simulink model "plant_n"  (R2023a)
settings: Solver=FixedStepAuto  StartTime=0.0  StopTime=200  FixedStep=0.01  RelTol=1e-3
values from neighbouring files (symbols this model uses):
  filter_3 = conv([0.1,1],conv([0.1 1],[0.1 1]))    [main_proj.m]
  filter_x = conv([0.7,1],conv([0.7 1],[0.7 1]))    [main_proj.m]
  kd = 1.117    [main_proj.m]
  ki = 4.47    [main_proj.m]
  kp = 5.366    [main_proj.m]
libraries: neural x772, slpidlib x6
(part 1 of 26)
settings Model: Creator=Alex  LastModifiedBy=Alex

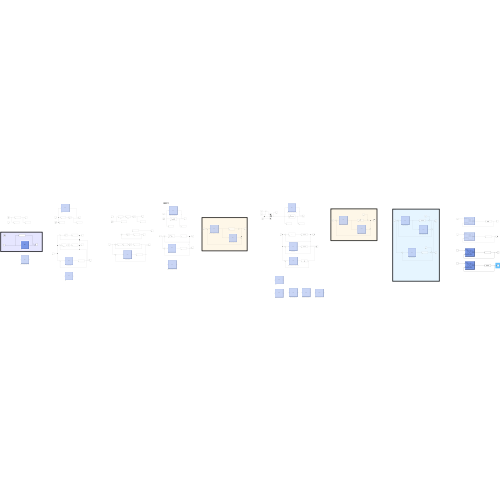
[thumbnail: Simulink's stored preview of the top-level diagram]
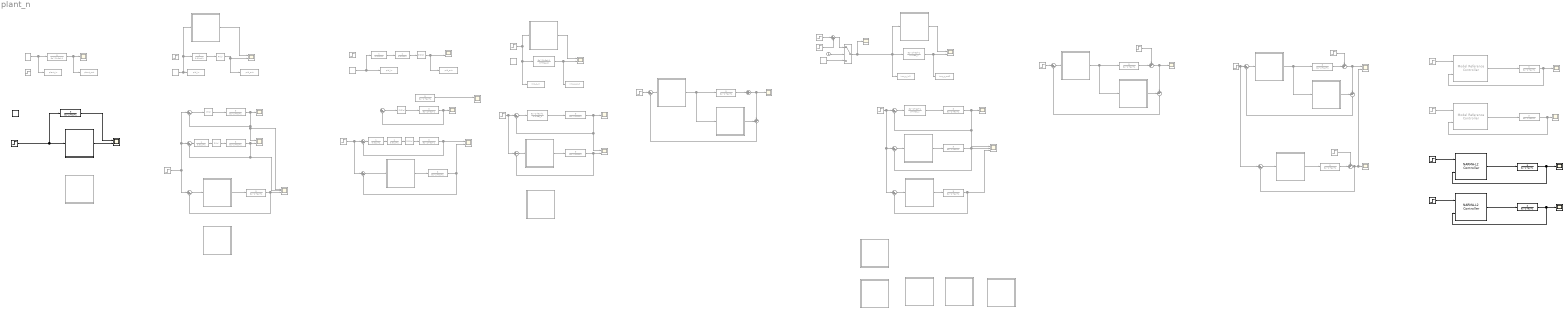
== system plant_n ==
  note: IMC1
  note: IMC1
  note: #2-3
  note: IMC2
  note: Compare
  Clock : Clock  Commented=on
  Filter{,1..5} (6 alike) : TransferFcn  Commented=on  Denominator=[0.01 1]
  Hr2 Neural Network : Subsystem  Commented=on  mask{pi_input_1_delayed_1=0, pi_input_1_delayed_2=0, pi_input_1_delayed_3=0, pi_input_1_delayed_4=0, pi_input_1_delayed_5=0, pi_input_1_delayed_6=0, ai_layer_2_delayed_1=0, ai_layer_2_delayed_2=0, ai_layer_2_delayed_3=0, ai_layer_2_delayed_4=0, ai_layer_2_delayed_5=0, ai_layer_2_delayed_6=0}
      mask prompts: pi_input_1_delayed_1 "Preprocessed initial input 1 state at timestep 0."; pi_input_1_delayed_2 "Preprocessed initial input 1 state at timestep -1."; pi_input_1_delayed_3 "Preprocessed initial input 1 state at timestep -2."; pi_input_1_delayed_4 "Preprocessed initial input 1 state at timestep -3."; pi_input_1_delayed_5 "Preprocessed initial input 1 state at timestep -4."; pi_input_1_delayed_6 "Preprocessed initial input 1 state at timestep -5."; ai_layer_2_delayed_1 "Initial layer 2 state at timestep 0."; ai_layer_2_delayed_2 "Initial layer 2 state at timestep -1."; ai_layer_2_delayed_3 "Initial layer 2 state at timestep -2."; ai_layer_2_delayed_4 "Initial layer 2 state at timestep -3."; ai_layer_2_delayed_5 "Initial layer 2 state at timestep -4."; ai_layer_2_delayed_6 "Initial layer 2 state at timestep -5."
      mask help: NARX Neural Network
      mask Display: e = 0.06;c1 = [120 150 230]/255;c2 = ([120 150 230]+0)/383;c3 = ([120 150 230]+128)/383;patch([0 1 1 0],[0 0 1 1],c1);patch([0 1 1 1-e 1-e 0+e],[0 0 1 1-e 0+e 0+e],c2);patch([0 0 1 1-e 0+e 0+e],[0 1 1 1-e 1-e 0+e],c3);plot([0 1 1 0 0],[0 0 1 1 0]);fprintf('NNET');port_label('input',1,' x');port_label('output',1,'y ');
  Hr2 Neural Network1 : Subsystem  Commented=on  mask{pi_input_1_delayed_1=0, pi_input_1_delayed_2=0, pi_input_1_delayed_3=0, pi_input_1_delayed_4=0, pi_input_1_delayed_5=0, pi_input_1_delayed_6=0, ai_layer_2_delayed_1=0, ai_layer_2_delayed_2=0, ai_layer_2_delayed_3=0, ai_layer_2_delayed_4=0, ai_layer_2_delayed_5=0, ai_layer_2_delayed_6=0}
      mask prompts: pi_input_1_delayed_1 "Preprocessed initial input 1 state at timestep 0."; pi_input_1_delayed_2 "Preprocessed initial input 1 state at timestep -1."; pi_input_1_delayed_3 "Preprocessed initial input 1 state at timestep -2."; pi_input_1_delayed_4 "Preprocessed initial input 1 state at timestep -3."; pi_input_1_delayed_5 "Preprocessed initial input 1 state at timestep -4."; pi_input_1_delayed_6 "Preprocessed initial input 1 state at timestep -5."; ai_layer_2_delayed_1 "Initial layer 2 state at timestep 0."; ai_layer_2_delayed_2 "Initial layer 2 state at timestep -1."; ai_layer_2_delayed_3 "Initial layer 2 state at timestep -2."; ai_layer_2_delayed_4 "Initial layer 2 state at timestep -3."; ai_layer_2_delayed_5 "Initial layer 2 state at timestep -4."; ai_layer_2_delayed_6 "Initial layer 2 state at timestep -5."
      mask help: NARX Neural Network
      mask Display: e = 0.06;c1 = [120 150 230]/255;c2 = ([120 150 230]+0)/383;c3 = ([120 150 230]+128)/383;patch([0 1 1 0],[0 0 1 1],c1);patch([0 1 1 1-e 1-e 0+e],[0 0 1 1-e 0+e 0+e],c2);patch([0 0 1 1-e 0+e 0+e],[0 1 1 1-e 1-e 0+e],c3);plot([0 1 1 0 0],[0 0 1 1 0]);fprintf('NNET');port_label('input',1,' x');port_label('output',1,'y ');
  Model Reference Controller : neural/Control Systems/Model Reference Controller  Commented=on  Nrc=2  Nic=1  Njc=2  IW_y=[1.3296070716326384709 -0.36667365564127274435;-0.92185323515790129623 0.32176549306151730478;1.8261953391711005512 1.1281754253248745812;2.081392820408017208 2.4865299205213595712;-1.4909287274670399714 0.11639212606746167367;0.46823572131003837749 0.088058028945422958667;-3.7167881282734223092 -3.6115499799353769639;1.4818494564283275494 2.7065106913308607517;1.6336147121001232119 0.5526617491453283959;-1.4099156717193841448 1.1569049865994305293;2.3686870848592893601 0.25288849028859083923;2.2287742825271403824 1.4983710960221059416;-0.99597562651575011206 0.092697495980983160568]  IW_u=[1.4743410646594798941;-0.73002540571032126238;-3.0820427704285724424;0.53364081831524945443;1.3844574682777242014;2.2994849637659218189;2.6080515112590818561;3.3191492457743909661;1.1600250344356883847;-0.81107387337725145304;-1.7263490679486648283;1.3637884727556424114;3.5961364066710643783]  IW_r=[0.45584496253579021019 0.013979066064819245518;-0.83540458064475398015 1.3369817271325503683;-0.49045911110561435375 -0.06578369498370542634;0.44086030026716438446 1.2365458882040423205;0.69033400334907890628 2.4098721877448441298;1.5039634381991009437 0.51175229301770042145;1.9013613732802914225 1.6718666996047224504;-2.9483143371280129408 -1.2964596974028812504;-0.71195000730611490702 0.54602009870251633217;0.44073655635966751953 0.35072389102907663982;-1.2261650136974546754 1.134551000123763087;2.5679363865125237609 -0.10987449572256477448;2.2584822906744599358 -0.46293788513520239825]  B1_c=[-2.6017037059917864639;2.4831616770785935877;-0.69967804536117750303;1.8461053910394569222;2.0936927854540310356;-0.65037824755168882618;-2.2310647260244911294;-0.56723571538320094465;1.5155600736459127198;-1.1274619690803939775;1.1420008123431555358;1.7485537141513041171;-0.14304865642348835175]  B2_c=0.49859367527745002135  LW_c=[-0.21560786427349326599 0.42218755085198778065 -2.5168500644863760485 -4.3042775398034240908 3.0736528575785957429 1.2004145740052258873 4.8803098890969769386 -4.903765247557268836 -2.0021893479913686065 1.1830173515845407994 1.0326255901814056504 -3.0305678461035592264 3.5511257763553163436]  retraining_c=30  max_i_int=0.3  min_i_int=0.01  max_r_int=0.3  min_r_int=0.01  Ts=0.01  S1=15  Ni=7  Nj=7  sim_file=plant_daq  trainfun=trainlm  Use_validation=1  Use_Testing=1  Use_Inc_training=0  Use_previous_weights=1  max_i=11  min_i=-11  max_r=1  min_r=-1  sam_training=7000  sam_training_c=7000  epochs=1000  epochs_c=1000  minp=-10.988507742147215041  maxp=10.979768684749934948  mint=-3.8286854023162479876  maxt=10.979768684749934948  Normalize=0  IW=[-0.096196767151805792628 0.069688900253981111987 -0.11414632395728388503 0.03380310834462384173 -0.10394306603562472602 0.050369638603738324523 -0.20070416107256491833;0.085825298980490752343 -0.13125992720494794597 0.36917943697583388563 -0.19267163875602047463 -0.12007252442864312092 -0.24919086144928226378 0.30995091781594286129;-0.12454285491314218137 -0.18617550753854025802 0.18540473952509214928 0.20790267007548821065 -0.35324104140001583163 -0.16301940699644387744 0.091419463919828858334;-5.5119777850224693555e-06 -4.3359379370616243346e-06 -1.692030312561132975e-05 -2.2407042060184435114e-06 -3.0824615230320695153e-06 -5.1366564063586963562e-06 1.6545291798370634416e-05;0.0096957497798623153845 0.38050449051489737551 0.49944098399193459503 0.052421264870644052047 0.027626071015783241341 -0.36332086427729193279 0.46254873826058989783;-3.8688801806231596213e-06 -1.0783090112052266869e-05 -1.5675682343423281539e-05 -7.4352360639534707218e-06 -5.9748050151522376945e-07 6.9622726526791568717e-07 1.0233518157329770306e-05;0.23425627076448132802 0.10948830117755810332 -0.08580339920518249841 -0.21619749925114917222 0.16691984566404238777 0.15408819517119581866 -0.069656411359783024229;-0.17923481973226779163 -0.3734132355570558004 0.48772350790411489463 -0.43203311567451913033 -0.10549166178544495953 -0.30648285248500672928 -0.59056268250324595037;8.0890264109084130371e-06 2.9234435920443260661e-06 1.8712401957121897343e-05 4.0566587345294193853e-06 7.6631724295067294133e-06 4.2821287801742582337e-06 -1.2706017327725187095e-05;1.1731657906753173472e-05 3.1258156594595680033e-05 -2.6258343721541373811e-05 2.5941834218704739663e-05 3.5192148815632747459e-05 -1.5866530394084238777e-07 0.00020205172082766727042;-0.02178867318460908642 -0.046180440291236031503 0.39918583548546565654 -0.34835569987993630914 -0.10550563278802824185 0.087890029577883874157 -0.00071868845735556226382;-5.3490863767874186421e-06 1.4045185164832040231e-05 -7.6256354641288490573e-08 2.3169813635436790412e-05 9.8313534835968070677e-06 6.75036488191517481e-06 -3.6223838976722067928e-06;-0.13726365515915717186 -0.095200399053326764665 -0.15941322116255240982 -0.15519989652548507597 -0.2727743328836970127 -0.15191535413502202378 -0.16028878504460999932;4.6955858084253991781e-06 1.2494144626207117596e-05 2.2531800415098768612e-05 1.9874998297332325268e-05 1.3465405020560401939e-05 9.1194981327321660627e-06 -1.8127978044236095495e-05;0.14452980362769671241 0.24589824886465630471 -0.06728997165946196124 -0.36848294936000547395 0.44609571336419373555 0.054463981727507444763 -0.021044829830446871999]  LW1_2=[0.14861091555967201328 0.34478204326288452997 0.3558400654392538387 0.35697598455192458555 0.18931759569298736712 0.17768697107890479847 0.17484250964170391929;0.10845671338328814748 0.093852273917411035975 0.21262993797098922455 0.25596645909310122846 0.03588848686131131116 -0.0027870875718595650682 0.13757477966585121565;0.11305853539800223007 -0.022956663362413178009 -0.069931506800843312721 0.09056872955326833452 -0.26634262306463429848 -0.021395817519269735851 -0.060213873715242928475;-0.15751443709582305108 -0.071910990277698094708 -0.086889799389636174221 0.043642285196309575646 0.021412316354041019406 -0.072400345203477350919 0.10512459549057595609;0.07328804631452078 0.17655010165892379148 0.21608305921005074857 0.14019704406872546265 -0.055947104098045666309 -0.14050413984766549347 -0.093226998770194094424;-0.10510622413701710409 -0.17857341457355369041 -0.21175342224952389825 0.12384087263403595336 0.068551462408649635472 0.10542717481883989716 -0.052278576669757423345;0.40219978853351451287 0.22296679464031857187 0.086629644932335506113 0.19508328152199636008 0.15141128908754003524 0.12458706880442040055 0.14023376450104427238;0.25628758153926928243 0.031225546226214852263 0.11782935558514234797 -0.23477352793508235451 -0.083828567511907856047 -0.25982638796543844339 -0.52206284880918452096;0.17030504793840781086 -0.02282146268343115264 0.083332278259328915193 0.11274766977691731695 0.028008942808686963094 -0.13262802397932524356 -0.025987817220298640303;0.0013909556386246470141 -0.083944162297307875487 0.11416165722051400955 0.04503174071203613904 -0.016222085233587247438 -0.037851508521260145146 0.043883852338576209706;0.64338859202817155758 0.6069049622101665431 0.49482781974953338189 0.38092861839956104753 0.29936635549479845286 0.22447584828212094332 0.19832556440503684714;0.068099588807467331675 0.072886989778193606027 -0.046842170049774672913 0.12373706988639987525 0.073210516138228751148 0.019840758304241756793 -0.15112284703497128047;0.28530079493460919204 0.33352897749471643873 0.10596091581332371667 0.0081673522743460139073 -0.017924793149277910842 0.12694401087948753437 -0.16136418841880059705;0.11642274843054778444 0.074105109096394408685 0.20235896634193009658 0.064117488026009986091 0.067174660640691455371 -0.077247328396860881483 -0.14578664248330414077;0.12003642055096161445 0.13888883993104197967 -0.11461700992364382001 -0.02930468335981756961 -0.19856153368656631608 0.0011886279195888265706 0.043542482653592139152]  LW2_1=[2.9091369964157201417e-06 -4.982490516236027056e-07 2.1890174474829930097e-06 -1.9728504797983674734 4.5716472867947320439e-07 -2.3334531115296801573 1.7382211233921508508e-06 4.7947476269963953372e-07 1.7190835726656092941 0.34478029171984708734 1.3510932500906089613e-06 1.2961611279267415409 1.9243581832398390012e-07 1.6134907670415230552 -3.1166438708490552883e-07]  B1=[1.7599919863203818959;2.108950439047047265;-1.2438460982794550258;0.53137975245226265475;0.91534079280602331785;-1.5888464635450123552;0.16472279329593006447;-0.0052740078755131591937;0.43987823236520207093;-0.34798910200549881822;0.76614366739175909782;0.087377677109910692477;1.2250236794160234144;-1.7847295653767702994;1.0962552864357135718]  B2=-0.37049821391249010416  S1c=13  Limit_output=0  min_output=-Inf  max_output=Inf  Ref_file=plant_daq
  Model Reference Controller1 : neural/Control Systems/Model Reference Controller  Commented=on  Nrc=7  Nic=7  Njc=7  IW_y=[-0.79464365804059655662 2.1484289208379534486 -0.044058828691782764286 -0.55555029930154753437 0.14667675800761273419 -0.4998593842863771064 0.81760037507028937576;-0.50822875300918157748 2.2181376450204783879 -0.42167244747835475049 -0.29902593449001463322 -2.125871150656503783 0.78516582748504037959 1.6702949833661873136;-0.070765005759242105565 1.2920678968125940411 0.90102979767096025299 1.0629121027429389024 -1.1038347098122409662 0.35437754446880181947 -1.5771715103135977021;0.20035893611114768964 -0.31180057605711880564 0.39164566394444372266 0.39612969170590039969 -0.41988358450536272803 -0.88958503187141491075 0.38351147320604717095;2.6238955631780553901 1.020713444883172949 0.99528089323565560598 0.045885013142218197824 0.86257580732106031718 0.28593209208873221483 0.47598467130126537183;-0.908018037123925148 1.228672687674863262 1.2023133827892757974 -0.96324586010628365784 -0.23416497767522209683 -0.12030377795837121635 -2.0675291097116623718;0.41533816760960501346 1.204356107818106647 0.01159434788394533844 0.17161459624115493749 1.0833932327601196732 1.529215572556056113 -0.13706386246296575759;-0.064556661353543765003 -0.88185373801636079971 -0.53210826826102597398 -0.3325097069527609972 -0.9312611861847124306 -0.71537621530040673701 -0.56297725957146438347;-0.3809502627188977586 -0.048511592562543323637 -0.71007668745409202593 -0.75819499831548398117 -0.031970864755670569402 -0.35296129439212542422 0.26505860017945703788;0.46152317549439059174 -1.6398711064885695965 0.54509581562013931233 -1.6938106521984743758 1.2337208285092762239 0.94007539774479387251 -0.71754519717443598914;-0.45200266983948972355 -0.0020310715043803106994 -2.1412365469707972387 -1.1023368992508975062 -1.6456411759471558653 0.70947282774466524646 -0.82104091573131476878;1.440784748775796098 -1.8376441932409106617 -0.55802733008814597859 -1.3618093837889633235 -1.9462876638480970382 -1.0036783041272168138 -0.12925964135217293816;-3.1342382588361057394 0.23348267128798555481 1.7478155121978942166 1.8165006112541788319 1.6738819740403874103 -1.4876665851706096788 -0.034843311154762357518]  IW_u=[-0.046255761019912911003 -0.69316382330787451593 -2.0776116422897694669 2.0025391782464452284 0.82884703867980991099 -2.5345545337648101025 0.46483676510372634594;-1.7698055116264468367 0.55823382689578604499 -0.36222172411316938545 -0.84886802737270727892 -1.8704348024682473373 1.1675778338157212222 0.97042649669864233797;-0.61865639345771150648 -0.80009664451939610519 1.4828008331647803963 0.47946982574324098492 -0.062096969746902978826 -2.1534869140557741929 0.83631630912520360521;-0.34305322714585373411 0.21935422443825858263 -0.11107873573194788908 0.45343281669491186658 0.36560410361572254212 -0.60484871133168061075 -0.51724998798723098581;-1.698246540787204939 -1.0822797583998413629 -1.2286644225022205212 1.1908906271127284171 1.3755276454548930332 -0.97772466499820653851 -0.44514280923902338483;0.36739955600632534516 -2.7024617632602314643 2.069348460857868055 0.71735372553643550475 -0.30215575888751522449 -1.3502363387377538384 1.6741379896959451834;1.3955989494813125784 1.2551610081368647087 0.21374539754949020698 0.76971921192628633968 -0.48885298409161975774 1.2349374647710087416 -0.36214967283008642207;0.30687605029061820749 0.3340749626350684176 -0.64206263668083118912 -0.58224240252225567538 0.0075003573297177106305 0.24116026992893302427 0.54339263278813598745;-1.0941846471743050806 -0.29947237351847300069 1.2088917633251534678 1.5040390867711863621 -1.1777737411130877465 -1.3471081205938710834 -0.0055155550883392301387;0.51056230222148690778 1.7024944745959267323 2.22360325684208604 -0.029033522560449581684 -0.95559138542214294709 0.18241016017752773037 -2.4175017578863582379;-1.9120998149834671498 1.242736019551059945 0.046215507450039050585 0.48028837504460314412 -0.015238903065254064129 -0.75585853068115915754 1.26784955036653324;-0.90996572480345938594 1.3506677361330052811 -2.7953693629768685547 1.7007163529983533312 0.34799694797621832931 1.5590954486165662374 -2.5703506280917127746;1.4314988745733594477 -0.3673410534325072252 0.74129818813107550834 -3.5845617047176325798 -1.3292998408030021196 -0.35063405221730448158 -0.86072292592849997117]  IW_r=[0.73028570693971817107 0.058549062045015837219 0.0029509866742587209654 0.097140592551535467902 -0.36256195255076006934 -1.0096049928344204005 -0.40391358302102309263;-0.072696247559823040651 -0.37567110420201244025 0.28603043118168303138 -0.42885632484217905969 -0.51118851500734796556 0.096984857895986431586 0.24352873703067501321;0.35625699784972236772 0.24710787297601710666 -0.49219154496437872437 -0.83014548002746857414 -0.32866590319241412166 0.43124859267790649486 0.36371240264961446353;0.068338938837080226429 -0.099578054613466721046 0.35492550751387930141 -0.02540511665357805815 0.22168326265042775924 0.4251726530565569373 -0.1590544305219428467;0.26764399558122620171 0.56583249960290937786 0.76256268484367573102 -0.14843777561020274347 -0.1621082451476119346 -0.094171223778508797442 -0.1880283762014295923;0.61539505760708035353 -0.44890802888363728895 0.36153257937702609759 0.6296692793389193632 0.80053145240594636434 0.75470859068268270065 1.2428929384264653102;-0.31749780377910663542 0.37193244107229245232 0.43737111199078126944 0.032126629742241952226 0.86910924731010452682 -0.090515816492360623435 0.61071293287761252433;-0.41625349782449411196 -0.7048174179637791692 -0.32667230930724067139 -0.50925957833863477742 0.12508075561437959067 -0.2850646946403997406 -0.078634624858256063629;0.034683102804885485027 0.34637208381444622995 -0.56289598483515135285 -0.27836602966052081953 0.030827434069493481195 -0.59466260914215784972 0.32152674782100260087;-0.582733326001451446 -0.15949680560822759867 -0.2326356907827483167 -0.12192668243991111598 0.59505652179035029015 -0.78002904235134107314 -0.41473903203792883421;0.9444548655284901173 0.40137476472675098771 0.59055916251731410682 -0.15155965323419304247 0.60624981742513073257 -0.16924740176695995952 -0.021447259752632397145;1.3193284885647011961 0.41397484644954690713 0.55628871658105383258 1.5318941517995676715 0.89534445798256412363 1.1705885239740059234 1.2637311812647635811;0.30230504351222320381 -0.71372674616425457739 -0.070983080717408178484 -0.69243459918472172188 0.25838492465856244262 -0.99059473521888408154 0.26526518665238407735]  B1_c=[2.447341503863201595;-1.2710007411859902682;0.88006172193723308794;-0.7564947937481504292;-0.059194838985939135512;1.1718205023357561867;1.2811941109001756534;0.32369662991863046297;-0.58226220044045906565;-1.044212831891682125;-1.4306892641193809101;-1.8233287248740825959;-0.22382991475080094013]  B2_c=-0.14435919869938435012  LW_c=[0.79832781230902405412 1.8024028323230874005 1.1068785274746064662 -0.94627703437016663646 -1.3773810358647424756 -2.3582764471304802356 1.1419639984092126994 -0.63361895883095131765 -1.4289665500193884373 -0.26669125405834648301 0.032544600171880572193 -0.67553623828550124486 -1.9202703901294324584]  retraining_c=10  max_i_int=3  min_i_int=0.01  max_r_int=1  min_r_int=0.1  Ts=0.01  S1=13  Ni=6  Nj=6  sim_file=plant_daq  trainfun=trainlm  Use_validation=1  Use_Testing=1  Use_Inc_training=0  Use_previous_weights=1  max_i=11  min_i=-11  max_r=1  min_r=-1  sam_training=7000  sam_training_c=9000  epochs=3000  epochs_c=1000  minp=-10.626375356580251008  maxp=10.745194433269574574  mint=-13.263015560773336432  maxt=10.745194433269574574  Normalize=1  IW=[0.0016437995892085140517 -0.345155690308660279 -0.79815772333718804088 0.60372634155782167742 0.23415727532237209929 0.17792904012962298954;0.22957949750945919054 -0.15622237610174619094 0.24396763666340082199 0.26482402836072033159 -0.25604052039666530538 -0.30303858096957703161;-0.051155845306893689417 0.19126030750829633997 -0.66425174271758558042 0.8178920896634567228 -0.41526541475418410343 0.14169852757092696316;0.93058268867045867978 0.52372831281114595736 0.64810989140563279864 -0.1550302584936093242 -0.38941272523942838113 -0.25864079990157173849;0.016997734029832876207 -0.018555435660227645456 -0.047851948798315627198 0.067740759694393623547 -0.013850160712438962241 -0.0066796060868148897371;-0.066658648731238376306 0.066962251904906969213 0.14097519829332716412 -0.2391687794221788177 0.05722469548892866742 0.049391518627503801231;0.0108642242123012326 -0.0036614277987921475289 0.0083146311537025344857 0.022472585384539552761 -0.013672386052970093503 -0.02613174933738322131;-0.014549532425320581275 0.017551033762802585592 0.035625136819713430769 -0.050796587228074022158 0.0090912216196348816233 0.0043084733328543354039;0.13628034085508031192 -0.73697603295848368443 -0.86869164250847008546 -0.48744055029050703531 0.49237834376705952311 0.54163064437055474798;0.051505965683173948744 -0.050199536189684673682 -0.10813857577065597027 0.18192210271685291256 -0.044060540101279778435 -0.037760938304223452822;0.013715738882921515301 -0.014009726013654607082 -0.044220752348500945439 0.063708128500190419619 -0.01430379620039704848 -0.0076234535021776116473;-0.44740348194575774166 -0.14814695232318045304 -0.1461341622370314064 0.67190805162571942688 -0.54457650512616839755 0.012512326520960737053;0.59901363817764563535 0.81049651231320640754 -0.55550504407148215691 0.12810420772457126182 0.64338562151449485427 0.36922823925222358898]  LW1_2=[-0.30637727785622220766 0.41451943950801872774 -0.3168800724775626132 -0.17304755869815607872 0.52322073686537862169 0.80106748562568630412;0.42247781728233385623 0.60017438891460350714 -0.016930857165132470743 0.19874427120798807134 -0.74515127140598280686 0.59169017134439427785;0.28353089368412431881 0.66704440844547419065 -0.41735428066598462271 0.38959588295749009168 -0.055962625307553519327 0.81534024168910634867;0.57315734006341056972 0.87310373900666993219 -0.21840005854579075395 0.73712762347178839573 -0.10259198174531586334 -0.054739517338798074353;0.2057239510782008507 -0.058009739387542454125 -0.24674060762202731922 0.63845698701826880672 0.25961423345281831043 -0.55822970731722987292;-0.59858742011115639858 0.25800074756954977095 -0.077448108748316896177 -0.30397679131568655642 0.86679122177463419074 0.057871374789443243147;0.60687837105834596674 0.45690559030819138941 -0.29676882102437779354 -0.41585567592970068551 0.31137617952592844262 -0.56968706767279975178;0.13996733361262755913 -0.78344341488170721188 0.24081267052841975884 0.022365575027545814973 0.82516675682941986736 -0.66023801779109403398;0.39212321153227974735 0.60545111297687825846 -0.56430096927080097835 -0.30511734553815894611 -0.45153756243723497388 -0.30213917338428192272;0.44254778275896849982 -0.15534230864096335023 -0.54357634005032662294 0.64108636098550075832 0.10064699940144887502 -0.67529155261301387903;0.96239679642765219025 -0.38313263192835728121 -0.41032042458089884596 0.57835026479931261889 -0.71434174176655096389 0.24225809755906366205;-0.71075448443818201039 0.4685460115919310442 -0.3742983940457548786 0.094442705322269157597 0.49543185851447824053 0.48057463080634033048;-0.18631793129334295323 -0.78202714961397501447 0.42892471224436939936 -0.56889256525236153728 0.098925593853177340442 -0.016577889834103444466]  LW2_1=[8.9704576891283109878e-05 0.0017789834127241496015 -0.00064215861560980140327 7.8789369629780868373e-06 2.099274350584501736 0.58703873860536082141 0.93689969864882072237 -1.5663983371643550591 3.0010099968793004871e-05 -0.92037360538357015916 0.91619103332655993377 9.3837164808292097893e-06 2.1670742865124617872e-06]  B1=[1.7085185822481785411;-1.5501223828041372776;-1.040571980015641218;-0.53226337808174162269;-0.63469644712038730816;0.72610443775071498163;-0.015219606278969172522;-0.53478778587897957131;0.30427938511600427507;0.60338600510193918236;0.95632140334126136683;-1.6835062040842629916;-1.6896862583930678525]  B2=-0.12069960689370959339  S1c=13  Limit_output=0  min_output=-Inf  max_output=Inf  Ref_file=plant_daq
  NARMA-L2 Controller : neural/Control Systems/NARMA-L2 Controller  Normalize=1  IW1_1=[1.1571738728005476204 0.93117029394905481698 0.84286216680037950866 0.39375060879211809528 0.59814436725544450901;-0.50014757697291112315 1.1213827677607333122 -0.41626610533667884884 -0.28421885879757785576 0.3056781357632270546;0.65643020805698770737 -0.60847058264088915713 0.25132547300992058581 -0.022738032737888776158 0.015304676296251078921;0.21715636532568527439 0.86614123148494504001 -0.57181113229249114216 0.12865018808853009857 -0.10353171227824382872;0.7090828828762359981 -1.3827734916489657913 1.0633248420960066394 -0.53227897134557722314 -0.18501845991713092299;-0.53875645023075358075 1.3369735720500766085 1.6039379388487560174 0.087932795626919885157 -1.0299135864558472964;-0.06608951253600182929 -0.19583781990660956152 0.042028814486793027172 0.55156890311502060342 -0.4863088962355333611;-0.71767320518037747146 0.23443192617377056619 0.059650652138784981959 -0.090850713494876972343 0.083377294987000694082;-0.025542026115630635935 1.4480173400602240896 0.69448008506947744856 1.4412153878887667968 0.63122792931272697636;-0.93174147644012450531 -0.10630386938765938598 -0.80067274674952482183 0.43173411600474320693 1.3401428172583864651;0.17197406797599856798 -1.3331625368641966123 0.72509006478496118575 -0.14091605094824946609 0.10755390845008463985;0.77970651587174966135 -1.5496499844595486017 0.62611133329995916075 0.2910189882895093394 -0.36307554631556243629;1.1553326527551690539 1.6142820108522202283 0.33932683480603487158 0.69842495450821928671 -0.37074689350900774665;-1.063165590752993106 1.1014065940300872271 -0.41048416507059604097 0.27438680451645791614 -0.26786891920858008076;-0.0057693985217563224094 1.5190100322203272665 -0.15014861371812907032 0.79770771004312446273 0.76691555873221395334]  IW3_2=[-1.5412362223023483576 -0.63946159059526741508 1.3588720579001996036 -0.23112729889892463797 -0.97207535486499874189;0.31621752320124180136 -0.051986386372772204478 0.012312806464611107324 -1.4890459424232262986 0.96697480099612054261;-1.1742335554563168021 -0.38139670620150106783 0.6262570357291784573 -0.77835065877580089655 -1.5905754038112760451;0.21550160749891122958 -1.6365741320922004842 1.6396672461974211021 0.1138518289087352281 -0.25453032653351526093;-0.83217048042976027311 0.41836111829081440439 0.23407660463602858458 0.83747169986886504933 -1.4385888394402031043;0.078903424927637924591 0.28919104498390924007 -0.43348908832288163273 1.3849349618611404011 -1.4962925468786139049;1.2789286566858810712 -0.69106828797732700043 0.4760556037218144354 1.1910090227896066306 -0.93616837132286279122;-0.85075632265485745531 -1.4115666330205389745 -0.08232336962817804471 1.4510437874474351183 0.65700216795313237661;-1.1601465565741151398 1.066851061666344469 -0.7805571093986564124 -1.1471491239654634242 -1.1181920728706193913;1.143180991399306512 -1.5291912459498653298 -0.2899473283697034387 1.3350271111652669553 0.26220076795912328205;0.86809352934312389305 -0.77458170314309060522 0.24160562714299610443 -1.4927274694748593475 -1.4108455583311121373;0.090121540283586737408 1.2078037064505362519 -0.40039695545991604853 1.985216629794274823 0.65604156893867160427;0.044911269375993996544 2.2326345915910330575 -0.57393286697849899003 0.61433241804681393283 0.032243560661817355362;-1.6459916828107374887 0.34430039224946540344 1.024350402267460991 -1.0828126184846331714 -0.90311952654036131705;1.2177261779806083375 0.53674220878032230519 -0.2475644182941683924 -1.2608914010231020431 1.1086650846219019417]  IW5_3=0.44545743977803392566  LW2_1=[3.2192828319514357619e-05 0.73439124755107831888 1.0045999297963998931 1.5746439900482043228 -0.0028336980708160907846 -2.0681837877014275039e-05 -0.13033365535756510911 -2.1413212936992014335 1.7222880985688209868e-06 -3.1238445994021751351e-05 -2.2077141730562961364 -0.63349921453416546679 6.7379331276970122933e-05 -1.201476937740369344 1.6988381665592116405e-05]  LW4_3=[0.24822241153672661151 1.6097621187972639412 0.02522071734930905057 0.98209129731003363961 -0.8937174987490476008 -0.84364444246547498629 -0.10853160463464642249 0.00089614862535315786048 0.0029578607402914523609 0.00102025719048513667 -0.0073852839224200416898 0.0073877303158363218441 -0.025202649034552999929 -0.030094635880682226586 -0.25455443308805081326]  LW5_4=0.016118901095918940908  LW6_5=-0.36710611293718553583  LW6_2=0.52347788362527836181  B1=[-2.0115566360292587156;0.48711189683678379758;-1.06589808932553054;-1.2262954123689389085;-1.3919077167774969173;0.87503960769730759761;0.37347931702109371521;0.051564483363330276822;-0.40107203796785029226;-0.96135002814272108029;-1.0794806777859053959;1.1456958887390111812;1.5191342008487802584;-2.0709204320226897167;2.471292372576378682]  B2=-0.45626343447748113347  B3=[2.4451080788116605902;-2.3891575663017521336;1.7216825779007711716;-1.6221272135609792198;1.5960129123540047758;1.0446953047400662218;-0.16785984067187631474;0.75861972353940754221;-0.33270264734724791511;0.67820600309318423982;0.99705019149041296256;1.3214064331043711142;1.6568445474611861457;-1.9938238316331282629;2.8024110410756950529]  B4=-1.4672521537596843189  Limit_output=0  min_output=-Inf  max_output=Inf  Use_Previous_Weights=1  Ts=0.5  S1=15  Ni=3  Nj=3  sim_file=plant_daq  trainfun=trainlm  Use_validation=1  Use_Testing=1  max_i=5  min_i=-5  max_i_int=40  min_i_int=2  sam_training=3000  epochs=1000  minp=-4.9963437623669424426  maxp=4.9814320737441537545  mint=-14.871534131182201577  maxt=4.9814320737441537545
  NARMA-L2 Controller1 : neural/Control Systems/NARMA-L2 Controller  Normalize=0  IW1_1=[0.58191848450669592108 0.56649325403973671555 0.36092376067206544121;-0.58191727706747875537 -0.5664948105982277049 -0.36092420228434290985;0.11563301984396186228 -0.04772626566886339905 0.0025686828794067532306;-0.11418561502549451347 0.047240762917243321606 -0.0025117945950874870191;-0.76799272534250118127 -0.35464182611762656849 -0.70185342375687687078;-0.088812939295320442179 0.036744067978180521006 -0.0019538784291780663879;-0.099224468151080907896 0.041042426816029244085 -0.0021847885678526923932;0.10533394867931342165 -0.043572866330174417349 0.0023189162342712784509;-0.11632610645248886438 0.048281081685838680984 -0.0025255181832816967109;-0.3747398033229438763 0.15866046268301473021 -0.0073480424523610027646]  IW3_2=[0.017953985222737015026 -0.018996023712122299398 -0.0013818555138843599539;-0.00053339699488158824527 0.0019955666421455648535 -0.00078712028271797249927;0.22874790380353882124 -0.19107844073483506997 0.47636172455621283994;0.10290028100784597009 -0.2599252236234735336 0.16975691446972998588;-0.00029488129775476532675 0.00039091972336983006175 2.5327455080752592025e-05;0.022332676810695631375 -0.21105327450690677948 -0.063316214074804241796;0.055862421330756042992 0.13430109265806933205 -0.20608758420312636717;7.209760391719503142e-05 -0.00013946980093046474811 2.9117458590862118842e-05;0.037857913385947829232 -0.037050197509928640971 0.00078209690007195915851;0.094445547903565407744 -0.095287219707146486591 -0.0013477064263671886812]  IW5_3=-0.60941188926541967064  LW2_1=[-0.41277567813239390837 -0.41277518623268311115 -1.6027772038279322064 0.91213166172522108788 -1.3332092952025119675e-07 2.4614621716782014715 1.6671065133738278696 -2.8512645229995579044 0.74811079864707730191 0.00087497549664910709809]  LW4_3=[-1.4051220687038403767 0.48277695227515371457 -3.6536688476148451484e-06 6.2226804406700317882e-05 -0.63565132415438363456 -1.0205012571849765145e-05 5.446434288244276779e-05 0.56229201454950594741 0.40165888934245902453 -0.34337306656137434047]  LW5_4=0.050862400088725168157  LW6_5=-0.52420416064757524577  LW6_2=-3.9080794985166900091  B1=[-2.7328399138853218808;2.7328420061741960367;2.2041274484062842731;0.72612464107691987447;0.082966113225345972104;-0.050453355012969346161;-0.88227980572659048253;-1.6281133068905027095;-1.8204648885387884061;2.5484949110808581274]  B2=0.37105250951788820712  B3=[-2.8720677033642361131;2.1405869715848999668;1.5007642979134911965;-0.88797620970999235901;0.094454483073317205277;0.3051144079482732141;0.92935056270180094184;1.6059627065840529347;2.622595087742555453;3.2978398539803608358]  B4=0.16960012538424493189  Limit_output=0  min_output=-Inf  max_output=Inf  Use_Previous_Weights=1  Ts=0.5  S1=10  Ni=2  Nj=2  sim_file=plant_daq  trainfun=trainlm  Use_validation=1  Use_Testing=1  max_i=10  min_i=-10  max_i_int=2  min_i_int=0.1  sam_training=2000  epochs=4000  minp=-9.9895524928611045823  maxp=9.9816078952272135894  mint=-17.670030440875180489  maxt=9.9816078952272135894
  NARX Neural Network : Subsystem  Commented=on  mask{pi_input_1_delayed_1=0, pi_input_1_delayed_2=0, pi_input_1_delayed_3=0, pi_input_1_delayed_4=0, pi_input_1_delayed_5=0, pi_input_1_delayed_6=0, pi_input_1_delayed_7=0, pi_input_1_delayed_8=0, pi_input_1_delayed_9=0, ai_layer_2_delayed_1=0, ai_layer_2_delayed_2=0, ai_layer_2_delayed_3=0, ai_layer_2_delayed_4=0, ai_layer_2_delayed_5=0, ai_layer_2_delayed_6=0, ai_layer_2_delayed_7=0, ai_layer_2_delayed_8=0, ai_layer_2_delayed_9=0}
      mask prompts: pi_input_1_delayed_1 "Preprocessed initial input 1 state at timestep 0."; pi_input_1_delayed_2 "Preprocessed initial input 1 state at timestep -1."; pi_input_1_delayed_3 "Preprocessed initial input 1 state at timestep -2."; pi_input_1_delayed_4 "Preprocessed initial input 1 state at timestep -3."; pi_input_1_delayed_5 "Preprocessed initial input 1 state at timestep -4."; pi_input_1_delayed_6 "Preprocessed initial input 1 state at timestep -5."; pi_input_1_delayed_7 "Preprocessed initial input 1 state at timestep -6."; pi_input_1_delayed_8 "Preprocessed initial input 1 state at timestep -7."; pi_input_1_delayed_9 "Preprocessed initial input 1 state at timestep -8."; ai_layer_2_delayed_1 "Initial layer 2 state at timestep 0."; ai_layer_2_delayed_2 "Initial layer 2 state at timestep -1."; ai_layer_2_delayed_3 "Initial layer 2 state at timestep -2."; ai_layer_2_delayed_4 "Initial layer 2 state at timestep -3."; ai_layer_2_delayed_5 "Initial layer 2 state at timestep -4."; ai_layer_2_delayed_6 "Initial layer 2 state at timestep -5."; ai_layer_2_delayed_7 "Initial layer 2 state at timestep -6."; ai_layer_2_delayed_8 "Initial layer 2 state at timestep -7."; ai_layer_2_delayed_9 "Initial layer 2 state at timestep -8."
      mask help: NARX Neural Network
      mask Display: e = 0.06;c1 = [120 150 230]/255;c2 = ([120 150 230]+0)/383;c3 = ([120 150 230]+128)/383;patch([0 1 1 0],[0 0 1 1],c1);patch([0 1 1 1-e 1-e 0+e],[0 0 1 1-e 0+e 0+e],c2);patch([0 0 1 1-e 0+e 0+e],[0 1 1 1-e 1-e 0+e],c3);plot([0 1 1 0 0],[0 0 1 1 0]);fprintf('NNET');port_label('input',1,' x');port_label('output',1,'y ');
  NARX Neural Network Best : Subsystem  Commented=on  mask{pi_input_1_delayed_1=0, pi_input_1_delayed_2=0, pi_input_1_delayed_3=0, pi_input_1_delayed_4=0, ai_layer_2_delayed_1=0, ai_layer_2_delayed_2=0, ai_layer_2_delayed_3=0, ai_layer_2_delayed_4=0}
      mask prompts: pi_input_1_delayed_1 "Preprocessed initial input 1 state at timestep 0."; pi_input_1_delayed_2 "Preprocessed initial input 1 state at timestep -1."; pi_input_1_delayed_3 "Preprocessed initial input 1 state at timestep -2."; pi_input_1_delayed_4 "Preprocessed initial input 1 state at timestep -3."; ai_layer_2_delayed_1 "Initial layer 2 state at timestep 0."; ai_layer_2_delayed_2 "Initial layer 2 state at timestep -1."; ai_layer_2_delayed_3 "Initial layer 2 state at timestep -2."; ai_layer_2_delayed_4 "Initial layer 2 state at timestep -3."
      mask help: NARX Neural Network
      mask Display: e = 0.06;c1 = [120 150 230]/255;c2 = ([120 150 230]+0)/383;c3 = ([120 150 230]+128)/383;patch([0 1 1 0],[0 0 1 1],c1);patch([0 1 1 1-e 1-e 0+e],[0 0 1 1-e 0+e 0+e],c2);patch([0 0 1 1-e 0+e 0+e],[0 1 1 1-e 1-e 0+e],c3);plot([0 1 1 0 0],[0 0 1 1 0]);fprintf('NNET');port_label('input',1,' x');port_label('output',1,'y ');
  NARX Neural Network Best1 : Subsystem  Commented=on  mask{pi_input_1_delayed_1=0, pi_input_1_delayed_2=0, pi_input_1_delayed_3=0, pi_input_1_delayed_4=0, ai_layer_2_delayed_1=0, ai_layer_2_delayed_2=0, ai_layer_2_delayed_3=0, ai_layer_2_delayed_4=0}
      mask prompts: pi_input_1_delayed_1 "Preprocessed initial input 1 state at timestep 0."; pi_input_1_delayed_2 "Preprocessed initial input 1 state at timestep -1."; pi_input_1_delayed_3 "Preprocessed initial input 1 state at timestep -2."; pi_input_1_delayed_4 "Preprocessed initial input 1 state at timestep -3."; ai_layer_2_delayed_1 "Initial layer 2 state at timestep 0."; ai_layer_2_delayed_2 "Initial layer 2 state at timestep -1."; ai_layer_2_delayed_3 "Initial layer 2 state at timestep -2."; ai_layer_2_delayed_4 "Initial layer 2 state at timestep -3."
      mask help: NARX Neural Network
      mask Display: e = 0.06;c1 = [120 150 230]/255;c2 = ([120 150 230]+0)/383;c3 = ([120 150 230]+128)/383;patch([0 1 1 0],[0 0 1 1],c1);patch([0 1 1 1-e 1-e 0+e],[0 0 1 1-e 0+e 0+e],c2);patch([0 0 1 1-e 0+e 0+e],[0 1 1 1-e 1-e 0+e],c3);plot([0 1 1 0 0],[0 0 1 1 0]);fprintf('NNET');port_label('input',1,' x');port_label('output',1,'y ');
  NARX Neural Network IMC Controller : Subsystem  Commented=on  mask{pi_input_1_delayed_1=0, pi_input_1_delayed_2=0, pi_input_1_delayed_3=0, pi_input_1_delayed_4=0, ai_layer_2_delayed_1=0, ai_layer_2_delayed_2=0, ai_layer_2_delayed_3=0, ai_layer_2_delayed_4=0}
      mask prompts: pi_input_1_delayed_1 "Preprocessed initial input 1 state at timestep 0."; pi_input_1_delayed_2 "Preprocessed initial input 1 state at timestep -1."; pi_input_1_delayed_3 "Preprocessed initial input 1 state at timestep -2."; pi_input_1_delayed_4 "Preprocessed initial input 1 state at timestep -3."; ai_layer_2_delayed_1 "Initial layer 2 state at timestep 0."; ai_layer_2_delayed_2 "Initial layer 2 state at timestep -1."; ai_layer_2_delayed_3 "Initial layer 2 state at timestep -2."; ai_layer_2_delayed_4 "Initial layer 2 state at timestep -3."
      mask help: NARX Neural Network
      mask Display: e = 0.06;c1 = [120 150 230]/255;c2 = ([120 150 230]+0)/383;c3 = ([120 150 230]+128)/383;patch([0 1 1 0],[0 0 1 1],c1);patch([0 1 1 1-e 1-e 0+e],[0 0 1 1-e 0+e 0+e],c2);patch([0 0 1 1-e 0+e 0+e],[0 1 1 1-e 1-e 0+e],c3);plot([0 1 1 0 0],[0 0 1 1 0]);fprintf('NNET');port_label('input',1,' x');port_label('output',1,'y ');
  NARX Neural Network IMC m9 : Subsystem  Commented=on  mask{pi_input_1_delayed_1=0, pi_input_1_delayed_2=0, pi_input_1_delayed_3=0, pi_input_1_delayed_4=0, pi_input_1_delayed_5=0, pi_input_1_delayed_6=0, pi_input_1_delayed_7=0, pi_input_1_delayed_8=0, pi_input_1_delayed_9=0, ai_layer_2_delayed_1=0, ai_layer_2_delayed_2=0, ai_layer_2_delayed_3=0, ai_layer_2_delayed_4=0, ai_layer_2_delayed_5=0, ai_layer_2_delayed_6=0, ai_layer_2_delayed_7=0, ai_layer_2_delayed_8=0, ai_layer_2_delayed_9=0}
      mask prompts: pi_input_1_delayed_1 "Preprocessed initial input 1 state at timestep 0."; pi_input_1_delayed_2 "Preprocessed initial input 1 state at timestep -1."; pi_input_1_delayed_3 "Preprocessed initial input 1 state at timestep -2."; pi_input_1_delayed_4 "Preprocessed initial input 1 state at timestep -3."; pi_input_1_delayed_5 "Preprocessed initial input 1 state at timestep -4."; pi_input_1_delayed_6 "Preprocessed initial input 1 state at timestep -5."; pi_input_1_delayed_7 "Preprocessed initial input 1 state at timestep -6."; pi_input_1_delayed_8 "Preprocessed initial input 1 state at timestep -7."; pi_input_1_delayed_9 "Preprocessed initial input 1 state at timestep -8."; ai_layer_2_delayed_1 "Initial layer 2 state at timestep 0."; ai_layer_2_delayed_2 "Initial layer 2 state at timestep -1."; ai_layer_2_delayed_3 "Initial layer 2 state at timestep -2."; ai_layer_2_delayed_4 "Initial layer 2 state at timestep -3."; ai_layer_2_delayed_5 "Initial layer 2 state at timestep -4."; ai_layer_2_delayed_6 "Initial layer 2 state at timestep -5."; ai_layer_2_delayed_7 "Initial layer 2 state at timestep -6."; ai_layer_2_delayed_8 "Initial layer 2 state at timestep -7."; ai_layer_2_delayed_9 "Initial layer 2 state at timestep -8."
      mask help: NARX Neural Network
      mask Display: e = 0.06;c1 = [120 150 230]/255;c2 = ([120 150 230]+0)/383;c3 = ([120 150 230]+128)/383;patch([0 1 1 0],[0 0 1 1],c1);patch([0 1 1 1-e 1-e 0+e],[0 0 1 1-e 0+e 0+e],c2);patch([0 0 1 1-e 0+e 0+e],[0 1 1 1-e 1-e 0+e],c3);plot([0 1 1 0 0],[0 0 1 1 0]);fprintf('NNET');port_label('input',1,' x');port_label('output',1,'y ');
  NARX Neural Network IMC m9 copy : Subsystem  Commented=on  mask{pi_input_1_delayed_1=0, pi_input_1_delayed_2=0, pi_input_1_delayed_3=0, pi_input_1_delayed_4=0, pi_input_1_delayed_5=0, pi_input_1_delayed_6=0, pi_input_1_delayed_7=0, pi_input_1_delayed_8=0, pi_input_1_delayed_9=0, ai_layer_2_delayed_1=0, ai_layer_2_delayed_2=0, ai_layer_2_delayed_3=0, ai_layer_2_delayed_4=0, ai_layer_2_delayed_5=0, ai_layer_2_delayed_6=0, ai_layer_2_delayed_7=0, ai_layer_2_delayed_8=0, ai_layer_2_delayed_9=0}
      mask prompts: pi_input_1_delayed_1 "Preprocessed initial input 1 state at timestep 0."; pi_input_1_delayed_2 "Preprocessed initial input 1 state at timestep -1."; pi_input_1_delayed_3 "Preprocessed initial input 1 state at timestep -2."; pi_input_1_delayed_4 "Preprocessed initial input 1 state at timestep -3."; pi_input_1_delayed_5 "Preprocessed initial input 1 state at timestep -4."; pi_input_1_delayed_6 "Preprocessed initial input 1 state at timestep -5."; pi_input_1_delayed_7 "Preprocessed initial input 1 state at timestep -6."; pi_input_1_delayed_8 "Preprocessed initial input 1 state at timestep -7."; pi_input_1_delayed_9 "Preprocessed initial input 1 state at timestep -8."; ai_layer_2_delayed_1 "Initial layer 2 state at timestep 0."; ai_layer_2_delayed_2 "Initial layer 2 state at timestep -1."; ai_layer_2_delayed_3 "Initial layer 2 state at timestep -2."; ai_layer_2_delayed_4 "Initial layer 2 state at timestep -3."; ai_layer_2_delayed_5 "Initial layer 2 state at timestep -4."; ai_layer_2_delayed_6 "Initial layer 2 state at timestep -5."; ai_layer_2_delayed_7 "Initial layer 2 state at timestep -6."; ai_layer_2_delayed_8 "Initial layer 2 state at timestep -7."; ai_layer_2_delayed_9 "Initial layer 2 state at timestep -8."
      mask help: NARX Neural Network
      mask Display: e = 0.06;c1 = [120 150 230]/255;c2 = ([120 150 230]+0)/383;c3 = ([120 150 230]+128)/383;patch([0 1 1 0],[0 0 1 1],c1);patch([0 1 1 1-e 1-e 0+e],[0 0 1 1-e 0+e 0+e],c2);patch([0 0 1 1-e 0+e 0+e],[0 1 1 1-e 1-e 0+e],c3);plot([0 1 1 0 0],[0 0 1 1 0]);fprintf('NNET');port_label('input',1,' x');port_label('output',1,'y ');
  NARX Neural Network IMC m9 copy1 : Subsystem  Commented=on  mask{pi_input_1_delayed_1=0, pi_input_1_delayed_2=0, pi_input_1_delayed_3=0, pi_input_1_delayed_4=0, pi_input_1_delayed_5=0, pi_input_1_delayed_6=0, pi_input_1_delayed_7=0, pi_input_1_delayed_8=0, pi_input_1_delayed_9=0, ai_layer_2_delayed_1=0, ai_layer_2_delayed_2=0, ai_layer_2_delayed_3=0, ai_layer_2_delayed_4=0, ai_layer_2_delayed_5=0, ai_layer_2_delayed_6=0, ai_layer_2_delayed_7=0, ai_layer_2_delayed_8=0, ai_layer_2_delayed_9=0}
      mask prompts: pi_input_1_delayed_1 "Preprocessed initial input 1 state at timestep 0."; pi_input_1_delayed_2 "Preprocessed initial input 1 state at timestep -1."; pi_input_1_delayed_3 "Preprocessed initial input 1 state at timestep -2."; pi_input_1_delayed_4 "Preprocessed initial input 1 state at timestep -3."; pi_input_1_delayed_5 "Preprocessed initial input 1 state at timestep -4."; pi_input_1_delayed_6 "Preprocessed initial input 1 state at timestep -5."; pi_input_1_delayed_7 "Preprocessed initial input 1 state at timestep -6."; pi_input_1_delayed_8 "Preprocessed initial input 1 state at timestep -7."; pi_input_1_delayed_9 "Preprocessed initial input 1 state at timestep -8."; ai_layer_2_delayed_1 "Initial layer 2 state at timestep 0."; ai_layer_2_delayed_2 "Initial layer 2 state at timestep -1."; ai_layer_2_delayed_3 "Initial layer 2 state at timestep -2."; ai_layer_2_delayed_4 "Initial layer 2 state at timestep -3."; ai_layer_2_delayed_5 "Initial layer 2 state at timestep -4."; ai_layer_2_delayed_6 "Initial layer 2 state at timestep -5."; ai_layer_2_delayed_7 "Initial layer 2 state at timestep -6."; ai_layer_2_delayed_8 "Initial layer 2 state at timestep -7."; ai_layer_2_delayed_9 "Initial layer 2 state at timestep -8."
      mask help: NARX Neural Network
      mask Display: e = 0.06;c1 = [120 150 230]/255;c2 = ([120 150 230]+0)/383;c3 = ([120 150 230]+128)/383;patch([0 1 1 0],[0 0 1 1],c1);patch([0 1 1 1-e 1-e 0+e],[0 0 1 1-e 0+e 0+e],c2);patch([0 0 1 1-e 0+e 0+e],[0 1 1 1-e 1-e 0+e],c3);plot([0 1 1 0 0],[0 0 1 1 0]);fprintf('NNET');port_label('input',1,' x');port_label('output',1,'y ');
  NARX Neural Network imc 2nd Best : Subsystem  Commented=on  mask{pi_input_1_delayed_1=0, pi_input_1_delayed_2=0, pi_input_1_delayed_3=0, pi_input_1_delayed_4=0, ai_layer_2_delayed_1=0, ai_layer_2_delayed_2=0, ai_layer_2_delayed_3=0, ai_layer_2_delayed_4=0}
      mask prompts: pi_input_1_delayed_1 "Preprocessed initial input 1 state at timestep 0."; pi_input_1_delayed_2 "Preprocessed initial input 1 state at timestep -1."; pi_input_1_delayed_3 "Preprocessed initial input 1 state at timestep -2."; pi_input_1_delayed_4 "Preprocessed initial input 1 state at timestep -3."; ai_layer_2_delayed_1 "Initial layer 2 state at timestep 0."; ai_layer_2_delayed_2 "Initial layer 2 state at timestep -1."; ai_layer_2_delayed_3 "Initial layer 2 state at timestep -2."; ai_layer_2_delayed_4 "Initial layer 2 state at timestep -3."
      mask help: NARX Neural Network
      mask Display: e = 0.06;c1 = [120 150 230]/255;c2 = ([120 150 230]+0)/383;c3 = ([120 150 230]+128)/383;patch([0 1 1 0],[0 0 1 1],c1);patch([0 1 1 1-e 1-e 0+e],[0 0 1 1-e 0+e 0+e],c2);patch([0 0 1 1-e 0+e 0+e],[0 1 1 1-e 1-e 0+e],c3);plot([0 1 1 0 0],[0 0 1 1 0]);fprintf('NNET');port_label('input',1,' x');port_label('output',1,'y ');
  NARX Neural Network m8 : Subsystem  Commented=on  mask{pi_input_1_delayed_1=0, pi_input_1_delayed_2=0, pi_input_1_delayed_3=0, pi_input_1_delayed_4=0, pi_input_1_delayed_5=0, pi_input_1_delayed_6=0, pi_input_1_delayed_7=0, pi_input_1_delayed_8=0, pi_input_1_delayed_9=0, ai_layer_2_delayed_1=0, ai_layer_2_delayed_2=0, ai_layer_2_delayed_3=0, ai_layer_2_delayed_4=0, ai_layer_2_delayed_5=0, ai_layer_2_delayed_6=0, ai_layer_2_delayed_7=0, ai_layer_2_delayed_8=0, ai_layer_2_delayed_9=0}
      mask prompts: pi_input_1_delayed_1 "Preprocessed initial input 1 state at timestep 0."; pi_input_1_delayed_2 "Preprocessed initial input 1 state at timestep -1."; pi_input_1_delayed_3 "Preprocessed initial input 1 state at timestep -2."; pi_input_1_delayed_4 "Preprocessed initial input 1 state at timestep -3."; pi_input_1_delayed_5 "Preprocessed initial input 1 state at timestep -4."; pi_input_1_delayed_6 "Preprocessed initial input 1 state at timestep -5."; pi_input_1_delayed_7 "Preprocessed initial input 1 state at timestep -6."; pi_input_1_delayed_8 "Preprocessed initial input 1 state at timestep -7."; pi_input_1_delayed_9 "Preprocessed initial input 1 state at timestep -8."; ai_layer_2_delayed_1 "Initial layer 2 state at timestep 0."; ai_layer_2_delayed_2 "Initial layer 2 state at timestep -1."; ai_layer_2_delayed_3 "Initial layer 2 state at timestep -2."; ai_layer_2_delayed_4 "Initial layer 2 state at timestep -3."; ai_layer_2_delayed_5 "Initial layer 2 state at timestep -4."; ai_layer_2_delayed_6 "Initial layer 2 state at timestep -5."; ai_layer_2_delayed_7 "Initial layer 2 state at timestep -6."; ai_layer_2_delayed_8 "Initial layer 2 state at timestep -7."; ai_layer_2_delayed_9 "Initial layer 2 state at timestep -8."
      mask help: NARX Neural Network
      mask Display: e = 0.06;c1 = [120 150 230]/255;c2 = ([120 150 230]+0)/383;c3 = ([120 150 230]+128)/383;patch([0 1 1 0],[0 0 1 1],c1);patch([0 1 1 1-e 1-e 0+e],[0 0 1 1-e 0+e 0+e],c2);patch([0 0 1 1-e 0+e 0+e],[0 1 1 1-e 1-e 0+e],c3);plot([0 1 1 0 0],[0 0 1 1 0]);fprintf('NNET');port_label('input',1,' x');port_label('output',1,'y ');
  NARX Neural Network m8 gud (solution 2) : Subsystem  Commented=on  mask{pi_input_1_delayed_1=0, pi_input_1_delayed_2=0, pi_input_1_delayed_3=0, pi_input_1_delayed_4=0, pi_input_1_delayed_5=0, pi_input_1_delayed_6=0, pi_input_1_delayed_7=0, pi_input_1_delayed_8=0, pi_input_1_delayed_9=0, pi_input_1_delayed_10=0, pi_input_1_delayed_11=0, pi_input_1_delayed_12=0, ai_layer_2_delayed_1=0, ai_layer_2_delayed_2=0, ai_layer_2_delayed_3=0, ai_layer_2_delayed_4=0, ai_layer_2_delayed_5=0, ai_layer_2_delayed_6=0, ai_layer_2_delayed_7=0, ai_layer_2_delayed_8=0, ai_layer_2_delayed_9=0, ai_layer_2_delayed_10=0, ai_layer_2_delayed_11=0, ai_layer_2_delayed_12=0}
      mask prompts: pi_input_1_delayed_1 "Preprocessed initial input 1 state at timestep 0."; pi_input_1_delayed_2 "Preprocessed initial input 1 state at timestep -1."; pi_input_1_delayed_3 "Preprocessed initial input 1 state at timestep -2."; pi_input_1_delayed_4 "Preprocessed initial input 1 state at timestep -3."; pi_input_1_delayed_5 "Preprocessed initial input 1 state at timestep -4."; pi_input_1_delayed_6 "Preprocessed initial input 1 state at timestep -5."; pi_input_1_delayed_7 "Preprocessed initial input 1 state at timestep -6."; pi_input_1_delayed_8 "Preprocessed initial input 1 state at timestep -7."; pi_input_1_delayed_9 "Preprocessed initial input 1 state at timestep -8."; pi_input_1_delayed_10 "Preprocessed initial input 1 state at timestep -9."; pi_input_1_delayed_11 "Preprocessed initial input 1 state at timestep -10."; pi_input_1_delayed_12 "Preprocessed initial input 1 state at timestep -11."; ai_layer_2_delayed_1 "Initial layer 2 state at timestep 0."; ai_layer_2_delayed_2 "Initial layer 2 state at timestep -1."; ai_layer_2_delayed_3 "Initial layer 2 state at timestep -2."; ai_layer_2_delayed_4 "Initial layer 2 state at timestep -3."; ai_layer_2_delayed_5 "Initial layer 2 state at timestep -4."; ai_layer_2_delayed_6 "Initial layer 2 state at timestep -5."; ai_layer_2_delayed_7 "Initial layer 2 state at timestep -6."; ai_layer_2_delayed_8 "Initial layer 2 state at timestep -7."; ai_layer_2_delayed_9 "Initial layer 2 state at timestep -8."; ai_layer_2_delayed_10 "Initial layer 2 state at timestep -9."; ai_layer_2_delayed_11 "Initial layer 2 state at timestep -10."; ai_layer_2_delayed_12 "Initial layer 2 state at timestep -11."
      mask help: NARX Neural Network
      mask Display: e = 0.06;c1 = [120 150 230]/255;c2 = ([120 150 230]+0)/383;c3 = ([120 150 230]+128)/383;patch([0 1 1 0],[0 0 1 1],c1);patch([0 1 1 1-e 1-e 0+e],[0 0 1 1-e 0+e 0+e],c2);patch([0 0 1 1-e 0+e 0+e],[0 1 1 1-e 1-e 0+e],c3);plot([0 1 1 0 0],[0 0 1 1 0]);fprintf('NNET');port_label('input',1,' x');port_label('output',1,'y ');
  NARX Neural Network pretty gud : Subsystem  Commented=on  mask{pi_input_1_delayed_1=0, pi_input_1_delayed_2=0, pi_input_1_delayed_3=0, pi_input_1_delayed_4=0, pi_input_1_delayed_5=0, pi_input_1_delayed_6=0, pi_input_1_delayed_7=0, ai_layer_2_delayed_1=0, ai_layer_2_delayed_2=0, ai_layer_2_delayed_3=0, ai_layer_2_delayed_4=0, ai_layer_2_delayed_5=0, ai_layer_2_delayed_6=0, ai_layer_2_delayed_7=0}
      mask prompts: pi_input_1_delayed_1 "Preprocessed initial input 1 state at timestep 0."; pi_input_1_delayed_2 "Preprocessed initial input 1 state at timestep -1."; pi_input_1_delayed_3 "Preprocessed initial input 1 state at timestep -2."; pi_input_1_delayed_4 "Preprocessed initial input 1 state at timestep -3."; pi_input_1_delayed_5 "Preprocessed initial input 1 state at timestep -4."; pi_input_1_delayed_6 "Preprocessed initial input 1 state at timestep -5."; pi_input_1_delayed_7 "Preprocessed initial input 1 state at timestep -6."; ai_layer_2_delayed_1 "Initial layer 2 state at timestep 0."; ai_layer_2_delayed_2 "Initial layer 2 state at timestep -1."; ai_layer_2_delayed_3 "Initial layer 2 state at timestep -2."; ai_layer_2_delayed_4 "Initial layer 2 state at timestep -3."; ai_layer_2_delayed_5 "Initial layer 2 state at timestep -4."; ai_layer_2_delayed_6 "Initial layer 2 state at timestep -5."; ai_layer_2_delayed_7 "Initial layer 2 state at timestep -6."
      mask help: NARX Neural Network
      mask Display: e = 0.06;c1 = [120 150 230]/255;c2 = ([120 150 230]+0)/383;c3 = ([120 150 230]+128)/383;patch([0 1 1 0],[0 0 1 1],c1);patch([0 1 1 1-e 1-e 0+e],[0 0 1 1-e 0+e 0+e],c2);patch([0 0 1 1-e 0+e 0+e],[0 1 1 1-e 1-e 0+e],c3);plot([0 1 1 0 0],[0 0 1 1 0]);fprintf('NNET');port_label('input',1,' x');port_label('output',1,'y ');
  PI Neural Network : Subsystem  Commented=on  mask{pi_input_1_delayed_1=0, pi_input_1_delayed_2=0, pi_input_1_delayed_3=0, pi_input_1_delayed_4=0, pi_input_1_delayed_5=0, pi_input_1_delayed_6=0, pi_input_1_delayed_7=0, pi_input_1_delayed_8=0, pi_input_1_delayed_9=0, pi_input_1_delayed_10=0, pi_input_1_delayed_11=0, pi_input_1_delayed_12=0, ai_layer_2_delayed_1=0, ai_layer_2_delayed_2=0, ai_layer_2_delayed_3=0, ai_layer_2_delayed_4=0, ai_layer_2_delayed_5=0, ai_layer_2_delayed_6=0, ai_layer_2_delayed_7=0, ai_layer_2_delayed_8=0, ai_layer_2_delayed_9=0, ai_layer_2_delayed_10=0, ai_layer_2_delayed_11=0, ai_layer_2_delayed_12=0}
      mask prompts: pi_input_1_delayed_1 "Preprocessed initial input 1 state at timestep 0."; pi_input_1_delayed_2 "Preprocessed initial input 1 state at timestep -1."; pi_input_1_delayed_3 "Preprocessed initial input 1 state at timestep -2."; pi_input_1_delayed_4 "Preprocessed initial input 1 state at timestep -3."; pi_input_1_delayed_5 "Preprocessed initial input 1 state at timestep -4."; pi_input_1_delayed_6 "Preprocessed initial input 1 state at timestep -5."; pi_input_1_delayed_7 "Preprocessed initial input 1 state at timestep -6."; pi_input_1_delayed_8 "Preprocessed initial input 1 state at timestep -7."; pi_input_1_delayed_9 "Preprocessed initial input 1 state at timestep -8."; pi_input_1_delayed_10 "Preprocessed initial input 1 state at timestep -9."; pi_input_1_delayed_11 "Preprocessed initial input 1 state at timestep -10."; pi_input_1_delayed_12 "Preprocessed initial input 1 state at timestep -11."; ai_layer_2_delayed_1 "Initial layer 2 state at timestep 0."; ai_layer_2_delayed_2 "Initial layer 2 state at timestep -1."; ai_layer_2_delayed_3 "Initial layer 2 state at timestep -2."; ai_layer_2_delayed_4 "Initial layer 2 state at timestep -3."; ai_layer_2_delayed_5 "Initial layer 2 state at timestep -4."; ai_layer_2_delayed_6 "Initial layer 2 state at timestep -5."; ai_layer_2_delayed_7 "Initial layer 2 state at timestep -6."; ai_layer_2_delayed_8 "Initial layer 2 state at timestep -7."; ai_layer_2_delayed_9 "Initial layer 2 state at timestep -8."; ai_layer_2_delayed_10 "Initial layer 2 state at timestep -9."; ai_layer_2_delayed_11 "Initial layer 2 state at timestep -10."; ai_layer_2_delayed_12 "Initial layer 2 state at timestep -11."
      mask help: NARX Neural Network
      mask Display: e = 0.06;c1 = [120 150 230]/255;c2 = ([120 150 230]+0)/383;c3 = ([120 150 230]+128)/383;patch([0 1 1 0],[0 0 1 1],c1);patch([0 1 1 1-e 1-e 0+e],[0 0 1 1-e 0+e 0+e],c2);patch([0 0 1 1-e 0+e 0+e],[0 1 1 1-e 1-e 0+e],c3);plot([0 1 1 0 0],[0 0 1 1 0]);fprintf('NNET');port_label('input',1,' x');port_label('output',1,'y ');
  PI Neural Network backup : Subsystem  Commented=on  mask{pi_input_1_delayed_1=0, pi_input_1_delayed_2=0, pi_input_1_delayed_3=0, pi_input_1_delayed_4=0, pi_input_1_delayed_5=0, pi_input_1_delayed_6=0, pi_input_1_delayed_7=0, pi_input_1_delayed_8=0, pi_input_1_delayed_9=0, pi_input_1_delayed_10=0, pi_input_1_delayed_11=0, pi_input_1_delayed_12=0, ai_layer_2_delayed_1=0, ai_layer_2_delayed_2=0, ai_layer_2_delayed_3=0, ai_layer_2_delayed_4=0, ai_layer_2_delayed_5=0, ai_layer_2_delayed_6=0, ai_layer_2_delayed_7=0, ai_layer_2_delayed_8=0, ai_layer_2_delayed_9=0, ai_layer_2_delayed_10=0, ai_layer_2_delayed_11=0, ai_layer_2_delayed_12=0}
      mask prompts: pi_input_1_delayed_1 "Preprocessed initial input 1 state at timestep 0."; pi_input_1_delayed_2 "Preprocessed initial input 1 state at timestep -1."; pi_input_1_delayed_3 "Preprocessed initial input 1 state at timestep -2."; pi_input_1_delayed_4 "Preprocessed initial input 1 state at timestep -3."; pi_input_1_delayed_5 "Preprocessed initial input 1 state at timestep -4."; pi_input_1_delayed_6 "Preprocessed initial input 1 state at timestep -5."; pi_input_1_delayed_7 "Preprocessed initial input 1 state at timestep -6."; pi_input_1_delayed_8 "Preprocessed initial input 1 state at timestep -7."; pi_input_1_delayed_9 "Preprocessed initial input 1 state at timestep -8."; pi_input_1_delayed_10 "Preprocessed initial input 1 state at timestep -9."; pi_input_1_delayed_11 "Preprocessed initial input 1 state at timestep -10."; pi_input_1_delayed_12 "Preprocessed initial input 1 state at timestep -11."; ai_layer_2_delayed_1 "Initial layer 2 state at timestep 0."; ai_layer_2_delayed_2 "Initial layer 2 state at timestep -1."; ai_layer_2_delayed_3 "Initial layer 2 state at timestep -2."; ai_layer_2_delayed_4 "Initial layer 2 state at timestep -3."; ai_layer_2_delayed_5 "Initial layer 2 state at timestep -4."; ai_layer_2_delayed_6 "Initial layer 2 state at timestep -5."; ai_layer_2_delayed_7 "Initial layer 2 state at timestep -6."; ai_layer_2_delayed_8 "Initial layer 2 state at timestep -7."; ai_layer_2_delayed_9 "Initial layer 2 state at timestep -8."; ai_layer_2_delayed_10 "Initial layer 2 state at timestep -9."; ai_layer_2_delayed_11 "Initial layer 2 state at timestep -10."; ai_layer_2_delayed_12 "Initial layer 2 state at timestep -11."
      mask help: NARX Neural Network
      mask Display: e = 0.06;c1 = [120 150 230]/255;c2 = ([120 150 230]+0)/383;c3 = ([120 150 230]+128)/383;patch([0 1 1 0],[0 0 1 1],c1);patch([0 1 1 1-e 1-e 0+e],[0 0 1 1-e 0+e 0+e],c2);patch([0 0 1 1-e 0+e 0+e],[0 1 1 1-e 1-e 0+e],c3);plot([0 1 1 0 0],[0 0 1 1 0]);fprintf('NNET');port_label('input',1,' x');port_label('output',1,'y ');
  PI Neural Network1 : Subsystem  Commented=on  mask{pi_input_1_delayed_1=0, pi_input_1_delayed_2=0, pi_input_1_delayed_3=0, pi_input_1_delayed_4=0, pi_input_1_delayed_5=0, pi_input_1_delayed_6=0, pi_input_1_delayed_7=0, pi_input_1_delayed_8=0, pi_input_1_delayed_9=0, pi_input_1_delayed_10=0, pi_input_1_delayed_11=0, pi_input_1_delayed_12=0, ai_layer_2_delayed_1=0, ai_layer_2_delayed_2=0, ai_layer_2_delayed_3=0, ai_layer_2_delayed_4=0, ai_layer_2_delayed_5=0, ai_layer_2_delayed_6=0, ai_layer_2_delayed_7=0, ai_layer_2_delayed_8=0, ai_layer_2_delayed_9=0, ai_layer_2_delayed_10=0, ai_layer_2_delayed_11=0, ai_layer_2_delayed_12=0}
      mask prompts: pi_input_1_delayed_1 "Preprocessed initial input 1 state at timestep 0."; pi_input_1_delayed_2 "Preprocessed initial input 1 state at timestep -1."; pi_input_1_delayed_3 "Preprocessed initial input 1 state at timestep -2."; pi_input_1_delayed_4 "Preprocessed initial input 1 state at timestep -3."; pi_input_1_delayed_5 "Preprocessed initial input 1 state at timestep -4."; pi_input_1_delayed_6 "Preprocessed initial input 1 state at timestep -5."; pi_input_1_delayed_7 "Preprocessed initial input 1 state at timestep -6."; pi_input_1_delayed_8 "Preprocessed initial input 1 state at timestep -7."; pi_input_1_delayed_9 "Preprocessed initial input 1 state at timestep -8."; pi_input_1_delayed_10 "Preprocessed initial input 1 state at timestep -9."; pi_input_1_delayed_11 "Preprocessed initial input 1 state at timestep -10."; pi_input_1_delayed_12 "Preprocessed initial input 1 state at timestep -11."; ai_layer_2_delayed_1 "Initial layer 2 state at timestep 0."; ai_layer_2_delayed_2 "Initial layer 2 state at timestep -1."; ai_layer_2_delayed_3 "Initial layer 2 state at timestep -2."; ai_layer_2_delayed_4 "Initial layer 2 state at timestep -3."; ai_layer_2_delayed_5 "Initial layer 2 state at timestep -4."; ai_layer_2_delayed_6 "Initial layer 2 state at timestep -5."; ai_layer_2_delayed_7 "Initial layer 2 state at timestep -6."; ai_layer_2_delayed_8 "Initial layer 2 state at timestep -7."; ai_layer_2_delayed_9 "Initial layer 2 state at timestep -8."; ai_layer_2_delayed_10 "Initial layer 2 state at timestep -9."; ai_layer_2_delayed_11 "Initial layer 2 state at timestep -10."; ai_layer_2_delayed_12 "Initial layer 2 state at timestep -11."
      mask help: NARX Neural Network
      mask Display: e = 0.06;c1 = [120 150 230]/255;c2 = ([120 150 230]+0)/383;c3 = ([120 150 230]+128)/383;patch([0 1 1 0],[0 0 1 1],c1);patch([0 1 1 1-e 1-e 0+e],[0 0 1 1-e 0+e 0+e],c2);patch([0 0 1 1-e 0+e 0+e],[0 1 1 1-e 1-e 0+e],c3);plot([0 1 1 0 0],[0 0 1 1 0]);fprintf('NNET');port_label('input',1,' x');port_label('output',1,'y ');
  PID Controller : slpidlib/PID Controller  Commented=on  Controller=PI  Form=Ideal  TimeDomain=Continuous-time  UseExternalTs=off  SampleTime=-1  IntegratorMethod=Forward Euler  FilterMethod=Forward Euler  ControllerParametersSource=internal  P=kp  I=1/ki  UseKiTs=off  D=kd  N=100  UseFilter=on  TunerSelectOption=Transfer Function Based (PID Tuner App)  InitialConditionSource=internal  InitialConditionForIntegrator=0  InitialConditionForFilter=0  DifferentiatorICPrevScaledInput=0  ExternalReset=none  TrackingMode=off  Kt=1  LimitOutput=off  SatLimitsSource=internal  UpperSaturationLimit=inf  LowerSaturationLimit=-inf  LinearizeAsGain=on  AntiWindupMode=none  Kb=1  LimitIntegrator=off  UpperIntegratorSaturationLimit=inf  LowerIntegratorSaturationLimit=-inf  POutMin=[]  POutMax=[]  IOutMin=[]  IOutMax=[]  DOutMin=[]  DOutMax=[]  NOutMin=[]  NOutMax=[]  SumOutMin=[]  SumOutMax=[]  SaturationOutMin=[]  SaturationOutMax=[]  PParamMin=[]  PParamMax=[]  IParamMin=[]  IParamMax=[]  DParamMin=[]  DParamMax=[]  NParamMin=[]  NParamMax=[]  KbParamMin=[]  KbParamMax=[]  KtParamMin=[]  KtParamMax=[]  KbOutMin=[]  KbOutMax=[]  KtOutMin=[]  KtOutMax=[]  IntegratorOutMin=[]  IntegratorOutMax=[]  FilterOutMin=[]  FilterOutMax=[]  SumI1OutMin=[]  SumI1OutMax=[]  SumI2OutMin=[]  SumI2OutMax=[]  SumI3OutMin=[]  SumI3OutMax=[]  SumI4OutMin=[]  SumI4OutMax=[]  SumDOutMin=[]  SumDOutMax=[]  DifferentiatorOutMin=[]  DifferentiatorOutMax=[]  FilterDiffOutCoefMin=[]  FilterDiffOutCoefMax=[]  ReciprocalOutMin=[]  ReciprocalOutMax=[]  SumDenOutMin=[]  SumDenOutMax=[]  SumNumOutMin=[]  SumNumOutMax=[]  DivideOutMin=[]  DivideOutMax=[]  UdiffTsProdOutMin=[]  UdiffTsProdOutMax=[]  NTsProdOutMin=[]  NTsProdOutMax=[]  UintegralTsProdOutMin=[]  UintegralTsProdOutMax=[]  UngainTsProdOutMin=[]  UngainTsProdOutMax=[]  ClampingZeroOutDataTypeStr=Inherit: Inherit via back propagation  ClampingZeroOutMin=[]  ClampingZeroOutMax=[]  FilterDenConstantOutDataTypeStr=Inherit: Inherit via back propagation  FilterDenConstantOutMin=[]  FilterDenConstantOutMax=[]  PCopyOutDataTypeStr=Inherit: Inherit via back propagation  PCopyOutMin=[]  PCopyOutMax=[]  NCopyOutDataTypeStr=Inherit: Inherit via back propagation  NCopyOutMin=[]  NCopyOutMax=[]  IntegratorContinuousStateAttributes=''  IntegratorStateMustResolveToSignalObject=off  IntegratorRTWStateStorageClass=Auto  FilterContinuousStateAttributes=''  FilterStateMustResolveToSignalObject=off  FilterRTWStateStorageClass=Auto  ParallelPVariant=Passthrough  IdealPVariant=InternalParameters  IVariant=InternalParameters  DVariant=Disabled  IntegratorVariant=Continuous  SatVariant=Disabled  AWVariant=Passthrough  PCopyVariant=Disabled  TRVariant=Disabled  FdbkBlocksVariant=Forward  IdealPFdbkVariant=Disabled  SatFdbkVariant=Disabled  DerivativeFilterVariant=Disabled  NVariant=Disabled  NCopyVariant=Disabled_SignalSpec  FilterICVariant=Disabled  IntegratorICVariant=InternalICs  ExternalResetVariant=Disabled  TRSumVariant=Passthrough  SumFdbkVariant=Disabled  SumVariant=Sum_PI  TsampFilterVariant=InternalTs  TsampNgainVariant=Passthrough  TsampIntegralVariant=Disabled_SignalSpec  ExternalSaturationOutDataTypeStr=Inherit: Same as second input
  PID Controller1 : slpidlib/PID Controller  Commented=on  Controller=PI  Form=Ideal  TimeDomain=Continuous-time  UseExternalTs=off  SampleTime=-1  IntegratorMethod=Forward Euler  FilterMethod=Forward Euler  ControllerParametersSource=internal  P=kp  I=1/ki  UseKiTs=off  D=kd  N=100  UseFilter=on  TunerSelectOption=Transfer Function Based (PID Tuner App)  InitialConditionSource=internal  InitialConditionForIntegrator=0  InitialConditionForFilter=0  DifferentiatorICPrevScaledInput=0  ExternalReset=none  TrackingMode=off  Kt=1  LimitOutput=off  SatLimitsSource=internal  UpperSaturationLimit=inf  LowerSaturationLimit=-inf  LinearizeAsGain=on  AntiWindupMode=none  Kb=1  LimitIntegrator=off  UpperIntegratorSaturationLimit=inf  LowerIntegratorSaturationLimit=-inf  POutMin=[]  POutMax=[]  IOutMin=[]  IOutMax=[]  DOutMin=[]  DOutMax=[]  NOutMin=[]  NOutMax=[]  SumOutMin=[]  SumOutMax=[]  SaturationOutMin=[]  SaturationOutMax=[]  PParamMin=[]  PParamMax=[]  IParamMin=[]  IParamMax=[]  DParamMin=[]  DParamMax=[]  NParamMin=[]  NParamMax=[]  KbParamMin=[]  KbParamMax=[]  KtParamMin=[]  KtParamMax=[]  KbOutMin=[]  KbOutMax=[]  KtOutMin=[]  KtOutMax=[]  IntegratorOutMin=[]  IntegratorOutMax=[]  FilterOutMin=[]  FilterOutMax=[]  SumI1OutMin=[]  SumI1OutMax=[]  SumI2OutMin=[]  SumI2OutMax=[]  SumI3OutMin=[]  SumI3OutMax=[]  SumI4OutMin=[]  SumI4OutMax=[]  SumDOutMin=[]  SumDOutMax=[]  DifferentiatorOutMin=[]  DifferentiatorOutMax=[]  FilterDiffOutCoefMin=[]  FilterDiffOutCoefMax=[]  ReciprocalOutMin=[]  ReciprocalOutMax=[]  SumDenOutMin=[]  SumDenOutMax=[]  SumNumOutMin=[]  SumNumOutMax=[]  DivideOutMin=[]  DivideOutMax=[]  UdiffTsProdOutMin=[]  UdiffTsProdOutMax=[]  NTsProdOutMin=[]  NTsProdOutMax=[]  UintegralTsProdOutMin=[]  UintegralTsProdOutMax=[]  UngainTsProdOutMin=[]  UngainTsProdOutMax=[]  ClampingZeroOutDataTypeStr=Inherit: Inherit via back propagation  ClampingZeroOutMin=[]  ClampingZeroOutMax=[]  FilterDenConstantOutDataTypeStr=Inherit: Inherit via back propagation  FilterDenConstantOutMin=[]  FilterDenConstantOutMax=[]  PCopyOutDataTypeStr=Inherit: Inherit via back propagation  PCopyOutMin=[]  PCopyOutMax=[]  NCopyOutDataTypeStr=Inherit: Inherit via back propagation  NCopyOutMin=[]  NCopyOutMax=[]  IntegratorContinuousStateAttributes=''  IntegratorStateMustResolveToSignalObject=off  IntegratorRTWStateStorageClass=Auto  FilterContinuousStateAttributes=''  FilterStateMustResolveToSignalObject=off  FilterRTWStateStorageClass=Auto  ParallelPVariant=Passthrough  IdealPVariant=InternalParameters  IVariant=InternalParameters  DVariant=Disabled  IntegratorVariant=Continuous  SatVariant=Disabled  AWVariant=Passthrough  PCopyVariant=Disabled  TRVariant=Disabled  FdbkBlocksVariant=Forward  IdealPFdbkVariant=Disabled  SatFdbkVariant=Disabled  DerivativeFilterVariant=Disabled  NVariant=Disabled  NCopyVariant=Disabled_SignalSpec  FilterICVariant=Disabled  IntegratorICVariant=InternalICs  ExternalResetVariant=Disabled  TRSumVariant=Passthrough  SumFdbkVariant=Disabled  SumVariant=Sum_PI  TsampFilterVariant=InternalTs  TsampNgainVariant=Passthrough  TsampIntegralVariant=Disabled_SignalSpec  ExternalSaturationOutDataTypeStr=Inherit: Same as second input
  PID Controller2 : slpidlib/PID Controller  Commented=on  Controller=PI  Form=Ideal  TimeDomain=Continuous-time  UseExternalTs=off  SampleTime=-1  IntegratorMethod=Forward Euler  FilterMethod=Forward Euler  ControllerParametersSource=internal  P=kp  I=1/ki  UseKiTs=off  D=kd  N=100  UseFilter=on  TunerSelectOption=Transfer Function Based (PID Tuner App)  InitialConditionSource=internal  InitialConditionForIntegrator=0  InitialConditionForFilter=0  DifferentiatorICPrevScaledInput=0  ExternalReset=none  TrackingMode=off  Kt=1  LimitOutput=off  SatLimitsSource=internal  UpperSaturationLimit=inf  LowerSaturationLimit=-inf  LinearizeAsGain=on  AntiWindupMode=none  Kb=1  LimitIntegrator=off  UpperIntegratorSaturationLimit=inf  LowerIntegratorSaturationLimit=-inf  POutMin=[]  POutMax=[]  IOutMin=[]  IOutMax=[]  DOutMin=[]  DOutMax=[]  NOutMin=[]  NOutMax=[]  SumOutMin=[]  SumOutMax=[]  SaturationOutMin=[]  SaturationOutMax=[]  PParamMin=[]  PParamMax=[]  IParamMin=[]  IParamMax=[]  DParamMin=[]  DParamMax=[]  NParamMin=[]  NParamMax=[]  KbParamMin=[]  KbParamMax=[]  KtParamMin=[]  KtParamMax=[]  KbOutMin=[]  KbOutMax=[]  KtOutMin=[]  KtOutMax=[]  IntegratorOutMin=[]  IntegratorOutMax=[]  FilterOutMin=[]  FilterOutMax=[]  SumI1OutMin=[]  SumI1OutMax=[]  SumI2OutMin=[]  SumI2OutMax=[]  SumI3OutMin=[]  SumI3OutMax=[]  SumI4OutMin=[]  SumI4OutMax=[]  SumDOutMin=[]  SumDOutMax=[]  DifferentiatorOutMin=[]  DifferentiatorOutMax=[]  FilterDiffOutCoefMin=[]  FilterDiffOutCoefMax=[]  ReciprocalOutMin=[]  ReciprocalOutMax=[]  SumDenOutMin=[]  SumDenOutMax=[]  SumNumOutMin=[]  SumNumOutMax=[]  DivideOutMin=[]  DivideOutMax=[]  UdiffTsProdOutMin=[]  UdiffTsProdOutMax=[]  NTsProdOutMin=[]  NTsProdOutMax=[]  UintegralTsProdOutMin=[]  UintegralTsProdOutMax=[]  UngainTsProdOutMin=[]  UngainTsProdOutMax=[]  ClampingZeroOutDataTypeStr=Inherit: Inherit via back propagation  ClampingZeroOutMin=[]  ClampingZeroOutMax=[]  FilterDenConstantOutDataTypeStr=Inherit: Inherit via back propagation  FilterDenConstantOutMin=[]  FilterDenConstantOutMax=[]  PCopyOutDataTypeStr=Inherit: Inherit via back propagation  PCopyOutMin=[]  PCopyOutMax=[]  NCopyOutDataTypeStr=Inherit: Inherit via back propagation  NCopyOutMin=[]  NCopyOutMax=[]  IntegratorContinuousStateAttributes=''  IntegratorStateMustResolveToSignalObject=off  IntegratorRTWStateStorageClass=Auto  FilterContinuousStateAttributes=''  FilterStateMustResolveToSignalObject=off  FilterRTWStateStorageClass=Auto  ParallelPVariant=Passthrough  IdealPVariant=InternalParameters  IVariant=InternalParameters  DVariant=Disabled  IntegratorVariant=Continuous  SatVariant=Disabled  AWVariant=Passthrough  PCopyVariant=Disabled  TRVariant=Disabled  FdbkBlocksVariant=Forward  IdealPFdbkVariant=Disabled  SatFdbkVariant=Disabled  DerivativeFilterVariant=Disabled  NVariant=Disabled  NCopyVariant=Disabled_SignalSpec  FilterICVariant=Disabled  IntegratorICVariant=InternalICs  ExternalResetVariant=Disabled  TRSumVariant=Passthrough  SumFdbkVariant=Disabled  SumVariant=Sum_PI  TsampFilterVariant=InternalTs  TsampNgainVariant=Passthrough  TsampIntegralVariant=Disabled_SignalSpec  ExternalSaturationOutDataTypeStr=Inherit: Same as second input
  PID Controller3 : slpidlib/PID Controller  Commented=on  Controller=PID  Form=Ideal  TimeDomain=Continuous-time  UseExternalTs=off  SampleTime=-1  IntegratorMethod=Forward Euler  FilterMethod=Forward Euler  ControllerParametersSource=internal  P=kp  I=1/ki  UseKiTs=off  D=kd  N=100  UseFilter=on  TunerSelectOption=Transfer Function Based (PID Tuner App)  InitialConditionSource=internal  InitialConditionForIntegrator=0  InitialConditionForFilter=0  DifferentiatorICPrevScaledInput=0  ExternalReset=none  TrackingMode=off  Kt=1  LimitOutput=off  SatLimitsSource=internal  UpperSaturationLimit=inf  LowerSaturationLimit=-inf  LinearizeAsGain=on  AntiWindupMode=none  Kb=1  LimitIntegrator=off  UpperIntegratorSaturationLimit=inf  LowerIntegratorSaturationLimit=-inf  POutMin=[]  POutMax=[]  IOutMin=[]  IOutMax=[]  DOutMin=[]  DOutMax=[]  NOutMin=[]  NOutMax=[]  SumOutMin=[]  SumOutMax=[]  SaturationOutMin=[]  SaturationOutMax=[]  PParamMin=[]  PParamMax=[]  IParamMin=[]  IParamMax=[]  DParamMin=[]  DParamMax=[]  NParamMin=[]  NParamMax=[]  KbParamMin=[]  KbParamMax=[]  KtParamMin=[]  KtParamMax=[]  KbOutMin=[]  KbOutMax=[]  KtOutMin=[]  KtOutMax=[]  IntegratorOutMin=[]  IntegratorOutMax=[]  FilterOutMin=[]  FilterOutMax=[]  SumI1OutMin=[]  SumI1OutMax=[]  SumI2OutMin=[]  SumI2OutMax=[]  SumI3OutMin=[]  SumI3OutMax=[]  SumI4OutMin=[]  SumI4OutMax=[]  SumDOutMin=[]  SumDOutMax=[]  DifferentiatorOutMin=[]  DifferentiatorOutMax=[]  FilterDiffOutCoefMin=[]  FilterDiffOutCoefMax=[]  ReciprocalOutMin=[]  ReciprocalOutMax=[]  SumDenOutMin=[]  SumDenOutMax=[]  SumNumOutMin=[]  SumNumOutMax=[]  DivideOutMin=[]  DivideOutMax=[]  UdiffTsProdOutMin=[]  UdiffTsProdOutMax=[]  NTsProdOutMin=[]  NTsProdOutMax=[]  UintegralTsProdOutMin=[]  UintegralTsProdOutMax=[]  UngainTsProdOutMin=[]  UngainTsProdOutMax=[]  ClampingZeroOutDataTypeStr=Inherit: Inherit via back propagation  ClampingZeroOutMin=[]  ClampingZeroOutMax=[]  FilterDenConstantOutDataTypeStr=Inherit: Inherit via back propagation  FilterDenConstantOutMin=[]  FilterDenConstantOutMax=[]  PCopyOutDataTypeStr=Inherit: Inherit via back propagation  PCopyOutMin=[]  PCopyOutMax=[]  NCopyOutDataTypeStr=Inherit: Inherit via back propagation  NCopyOutMin=[]  NCopyOutMax=[]  IntegratorContinuousStateAttributes=''  IntegratorStateMustResolveToSignalObject=off  IntegratorRTWStateStorageClass=Auto  FilterContinuousStateAttributes=''  FilterStateMustResolveToSignalObject=off  FilterRTWStateStorageClass=Auto  ParallelPVariant=Passthrough  IdealPVariant=InternalParameters  IVariant=InternalParameters  DVariant=InternalParameters  IntegratorVariant=Continuous  SatVariant=Disabled  AWVariant=Passthrough  PCopyVariant=Disabled  TRVariant=Disabled  FdbkBlocksVariant=Forward  IdealPFdbkVariant=Disabled  SatFdbkVariant=Disabled  DerivativeFilterVariant=ContFilter  NVariant=InternalParameters  NCopyVariant=Disabled  FilterICVariant=InternalICsFilter  IntegratorICVariant=InternalICs  ExternalResetVariant=Disabled  TRSumVariant=Passthrough  SumFdbkVariant=Disabled  SumVariant=Sum_PID  TsampFilterVariant=InternalTs  TsampNgainVariant=Passthrough  TsampIntegralVariant=Disabled_SignalSpec  ExternalSaturationOutDataTypeStr=Inherit: Same as second input
  PID Controller4 : slpidlib/PID Controller  Commented=on  Controller=PID  Form=Ideal  TimeDomain=Continuous-time  UseExternalTs=off  SampleTime=-1  IntegratorMethod=Forward Euler  FilterMethod=Forward Euler  ControllerParametersSource=internal  P=kp  I=1/ki  UseKiTs=off  D=kd  N=100  UseFilter=on  TunerSelectOption=Transfer Function Based (PID Tuner App)  InitialConditionSource=internal  InitialConditionForIntegrator=0  InitialConditionForFilter=0  DifferentiatorICPrevScaledInput=0  ExternalReset=none  TrackingMode=off  Kt=1  LimitOutput=off  SatLimitsSource=internal  UpperSaturationLimit=inf  LowerSaturationLimit=-inf  LinearizeAsGain=on  AntiWindupMode=none  Kb=1  LimitIntegrator=off  UpperIntegratorSaturationLimit=inf  LowerIntegratorSaturationLimit=-inf  POutMin=[]  POutMax=[]  IOutMin=[]  IOutMax=[]  DOutMin=[]  DOutMax=[]  NOutMin=[]  NOutMax=[]  SumOutMin=[]  SumOutMax=[]  SaturationOutMin=[]  SaturationOutMax=[]  PParamMin=[]  PParamMax=[]  IParamMin=[]  IParamMax=[]  DParamMin=[]  DParamMax=[]  NParamMin=[]  NParamMax=[]  KbParamMin=[]  KbParamMax=[]  KtParamMin=[]  KtParamMax=[]  KbOutMin=[]  KbOutMax=[]  KtOutMin=[]  KtOutMax=[]  IntegratorOutMin=[]  IntegratorOutMax=[]  FilterOutMin=[]  FilterOutMax=[]  SumI1OutMin=[]  SumI1OutMax=[]  SumI2OutMin=[]  SumI2OutMax=[]  SumI3OutMin=[]  SumI3OutMax=[]  SumI4OutMin=[]  SumI4OutMax=[]  SumDOutMin=[]  SumDOutMax=[]  DifferentiatorOutMin=[]  DifferentiatorOutMax=[]  FilterDiffOutCoefMin=[]  FilterDiffOutCoefMax=[]  ReciprocalOutMin=[]  ReciprocalOutMax=[]  SumDenOutMin=[]  SumDenOutMax=[]  SumNumOutMin=[]  SumNumOutMax=[]  DivideOutMin=[]  DivideOutMax=[]  UdiffTsProdOutMin=[]  UdiffTsProdOutMax=[]  NTsProdOutMin=[]  NTsProdOutMax=[]  UintegralTsProdOutMin=[]  UintegralTsProdOutMax=[]  UngainTsProdOutMin=[]  UngainTsProdOutMax=[]  ClampingZeroOutDataTypeStr=Inherit: Inherit via back propagation  ClampingZeroOutMin=[]  ClampingZeroOutMax=[]  FilterDenConstantOutDataTypeStr=Inherit: Inherit via back propagation  FilterDenConstantOutMin=[]  FilterDenConstantOutMax=[]  PCopyOutDataTypeStr=Inherit: Inherit via back propagation  PCopyOutMin=[]  PCopyOutMax=[]  NCopyOutDataTypeStr=Inherit: Inherit via back propagation  NCopyOutMin=[]  NCopyOutMax=[]  IntegratorContinuousStateAttributes=''  IntegratorStateMustResolveToSignalObject=off  IntegratorRTWStateStorageClass=Auto  FilterContinuousStateAttributes=''  FilterStateMustResolveToSignalObject=off  FilterRTWStateStorageClass=Auto  ParallelPVariant=Passthrough  IdealPVariant=InternalParameters  IVariant=InternalParameters  DVariant=InternalParameters  IntegratorVariant=Continuous  SatVariant=Disabled  AWVariant=Passthrough  PCopyVariant=Disabled  TRVariant=Disabled  FdbkBlocksVariant=Forward  IdealPFdbkVariant=Disabled  SatFdbkVariant=Disabled  DerivativeFilterVariant=ContFilter  NVariant=InternalParameters  NCopyVariant=Disabled  FilterICVariant=InternalICsFilter  IntegratorICVariant=InternalICs  ExternalResetVariant=Disabled  TRSumVariant=Passthrough  SumFdbkVariant=Disabled  SumVariant=Sum_PID  TsampFilterVariant=InternalTs  TsampNgainVariant=Passthrough  TsampIntegralVariant=Disabled_SignalSpec  ExternalSaturationOutDataTypeStr=Inherit: Same as second input
  PID Controller5 : slpidlib/PID Controller  Commented=on  Controller=PID  Form=Ideal  TimeDomain=Continuous-time  UseExternalTs=off  SampleTime=-1  IntegratorMethod=Forward Euler  FilterMethod=Forward Euler  ControllerParametersSource=internal  P=kp  I=1/ki  UseKiTs=off  D=kd  N=100  UseFilter=on  TunerSelectOption=Transfer Function Based (PID Tuner App)  InitialConditionSource=internal  InitialConditionForIntegrator=0  InitialConditionForFilter=0  DifferentiatorICPrevScaledInput=0  ExternalReset=none  TrackingMode=off  Kt=1  LimitOutput=off  SatLimitsSource=internal  UpperSaturationLimit=inf  LowerSaturationLimit=-inf  LinearizeAsGain=on  AntiWindupMode=none  Kb=1  LimitIntegrator=off  UpperIntegratorSaturationLimit=inf  LowerIntegratorSaturationLimit=-inf  POutMin=[]  POutMax=[]  IOutMin=[]  IOutMax=[]  DOutMin=[]  DOutMax=[]  NOutMin=[]  NOutMax=[]  SumOutMin=[]  SumOutMax=[]  SaturationOutMin=[]  SaturationOutMax=[]  PParamMin=[]  PParamMax=[]  IParamMin=[]  IParamMax=[]  DParamMin=[]  DParamMax=[]  NParamMin=[]  NParamMax=[]  KbParamMin=[]  KbParamMax=[]  KtParamMin=[]  KtParamMax=[]  KbOutMin=[]  KbOutMax=[]  KtOutMin=[]  KtOutMax=[]  IntegratorOutMin=[]  IntegratorOutMax=[]  FilterOutMin=[]  FilterOutMax=[]  SumI1OutMin=[]  SumI1OutMax=[]  SumI2OutMin=[]  SumI2OutMax=[]  SumI3OutMin=[]  SumI3OutMax=[]  SumI4OutMin=[]  SumI4OutMax=[]  SumDOutMin=[]  SumDOutMax=[]  DifferentiatorOutMin=[]  DifferentiatorOutMax=[]  FilterDiffOutCoefMin=[]  FilterDiffOutCoefMax=[]  ReciprocalOutMin=[]  ReciprocalOutMax=[]  SumDenOutMin=[]  SumDenOutMax=[]  SumNumOutMin=[]  SumNumOutMax=[]  DivideOutMin=[]  DivideOutMax=[]  UdiffTsProdOutMin=[]  UdiffTsProdOutMax=[]  NTsProdOutMin=[]  NTsProdOutMax=[]  UintegralTsProdOutMin=[]  UintegralTsProdOutMax=[]  UngainTsProdOutMin=[]  UngainTsProdOutMax=[]  ClampingZeroOutDataTypeStr=Inherit: Inherit via back propagation  ClampingZeroOutMin=[]  ClampingZeroOutMax=[]  FilterDenConstantOutDataTypeStr=Inherit: Inherit via back propagation  FilterDenConstantOutMin=[]  FilterDenConstantOutMax=[]  PCopyOutDataTypeStr=Inherit: Inherit via back propagation  PCopyOutMin=[]  PCopyOutMax=[]  NCopyOutDataTypeStr=Inherit: Inherit via back propagation  NCopyOutMin=[]  NCopyOutMax=[]  IntegratorContinuousStateAttributes=''  IntegratorStateMustResolveToSignalObject=off  IntegratorRTWStateStorageClass=Auto  FilterContinuousStateAttributes=''  FilterStateMustResolveToSignalObject=off  FilterRTWStateStorageClass=Auto  ParallelPVariant=Passthrough  IdealPVariant=InternalParameters  IVariant=InternalParameters  DVariant=InternalParameters  IntegratorVariant=Continuous  SatVariant=Disabled  AWVariant=Passthrough  PCopyVariant=Disabled  TRVariant=Disabled  FdbkBlocksVariant=Forward  IdealPFdbkVariant=Disabled  SatFdbkVariant=Disabled  DerivativeFilterVariant=ContFilter  NVariant=InternalParameters  NCopyVariant=Disabled  FilterICVariant=InternalICsFilter  IntegratorICVariant=InternalICs  ExternalResetVariant=Disabled  TRSumVariant=Passthrough  SumFdbkVariant=Disabled  SumVariant=Sum_PID  TsampFilterVariant=InternalTs  TsampNgainVariant=Passthrough  TsampIntegralVariant=Disabled_SignalSpec  ExternalSaturationOutDataTypeStr=Inherit: Same as second input
  PID Neural Network : Subsystem  Commented=on  mask{pi_input_1_delayed_1=0, pi_input_1_delayed_2=0, pi_input_1_delayed_3=0, pi_input_1_delayed_4=0, pi_input_1_delayed_5=0, pi_input_1_delayed_6=0, pi_input_1_delayed_7=0, ai_layer_2_delayed_1=0, ai_layer_2_delayed_2=0, ai_layer_2_delayed_3=0, ai_layer_2_delayed_4=0, ai_layer_2_delayed_5=0, ai_layer_2_delayed_6=0, ai_layer_2_delayed_7=0}
      mask prompts: pi_input_1_delayed_1 "Preprocessed initial input 1 state at timestep 0."; pi_input_1_delayed_2 "Preprocessed initial input 1 state at timestep -1."; pi_input_1_delayed_3 "Preprocessed initial input 1 state at timestep -2."; pi_input_1_delayed_4 "Preprocessed initial input 1 state at timestep -3."; pi_input_1_delayed_5 "Preprocessed initial input 1 state at timestep -4."; pi_input_1_delayed_6 "Preprocessed initial input 1 state at timestep -5."; pi_input_1_delayed_7 "Preprocessed initial input 1 state at timestep -6."; ai_layer_2_delayed_1 "Initial layer 2 state at timestep 0."; ai_layer_2_delayed_2 "Initial layer 2 state at timestep -1."; ai_layer_2_delayed_3 "Initial layer 2 state at timestep -2."; ai_layer_2_delayed_4 "Initial layer 2 state at timestep -3."; ai_layer_2_delayed_5 "Initial layer 2 state at timestep -4."; ai_layer_2_delayed_6 "Initial layer 2 state at timestep -5."; ai_layer_2_delayed_7 "Initial layer 2 state at timestep -6."
      mask help: NARX Neural Network
      mask Display: e = 0.06;c1 = [120 150 230]/255;c2 = ([120 150 230]+0)/383;c3 = ([120 150 230]+128)/383;patch([0 1 1 0],[0 0 1 1],c1);patch([0 1 1 1-e 1-e 0+e],[0 0 1 1-e 0+e 0+e],c2);patch([0 0 1 1-e 0+e 0+e],[0 1 1 1-e 1-e 0+e],c3);plot([0 1 1 0 0],[0 0 1 1 0]);fprintf('NNET');port_label('input',1,' x');port_label('output',1,'y ');
  PID Neural Network1 : Subsystem  Commented=on  mask{pi_input_1_delayed_1=0, pi_input_1_delayed_2=0, pi_input_1_delayed_3=0, pi_input_1_delayed_4=0, pi_input_1_delayed_5=0, pi_input_1_delayed_6=0, pi_input_1_delayed_7=0, ai_layer_2_delayed_1=0, ai_layer_2_delayed_2=0, ai_layer_2_delayed_3=0, ai_layer_2_delayed_4=0, ai_layer_2_delayed_5=0, ai_layer_2_delayed_6=0, ai_layer_2_delayed_7=0}
      mask prompts: pi_input_1_delayed_1 "Preprocessed initial input 1 state at timestep 0."; pi_input_1_delayed_2 "Preprocessed initial input 1 state at timestep -1."; pi_input_1_delayed_3 "Preprocessed initial input 1 state at timestep -2."; pi_input_1_delayed_4 "Preprocessed initial input 1 state at timestep -3."; pi_input_1_delayed_5 "Preprocessed initial input 1 state at timestep -4."; pi_input_1_delayed_6 "Preprocessed initial input 1 state at timestep -5."; pi_input_1_delayed_7 "Preprocessed initial input 1 state at timestep -6."; ai_layer_2_delayed_1 "Initial layer 2 state at timestep 0."; ai_layer_2_delayed_2 "Initial layer 2 state at timestep -1."; ai_layer_2_delayed_3 "Initial layer 2 state at timestep -2."; ai_layer_2_delayed_4 "Initial layer 2 state at timestep -3."; ai_layer_2_delayed_5 "Initial layer 2 state at timestep -4."; ai_layer_2_delayed_6 "Initial layer 2 state at timestep -5."; ai_layer_2_delayed_7 "Initial layer 2 state at timestep -6."
      mask help: NARX Neural Network
      mask Display: e = 0.06;c1 = [120 150 230]/255;c2 = ([120 150 230]+0)/383;c3 = ([120 150 230]+128)/383;patch([0 1 1 0],[0 0 1 1],c1);patch([0 1 1 1-e 1-e 0+e],[0 0 1 1-e 0+e 0+e],c2);patch([0 0 1 1-e 0+e 0+e],[0 1 1 1-e 1-e 0+e],c3);plot([0 1 1 0 0],[0 0 1 1 0]);fprintf('NNET');port_label('input',1,' x');port_label('output',1,'y ');
  Plant Neural Network 001 : Subsystem  mask{pi_input_1_delayed_1=0, pi_input_1_delayed_2=0, pi_input_1_delayed_3=0, pi_input_1_delayed_4=0, pi_input_1_delayed_5=0, ai_layer_2_delayed_1=0, ai_layer_2_delayed_2=0, ai_layer_2_delayed_3=0, ai_layer_2_delayed_4=0, ai_layer_2_delayed_5=0}
      mask prompts: pi_input_1_delayed_1 "Preprocessed initial input 1 state at timestep 0."; pi_input_1_delayed_2 "Preprocessed initial input 1 state at timestep -1."; pi_input_1_delayed_3 "Preprocessed initial input 1 state at timestep -2."; pi_input_1_delayed_4 "Preprocessed initial input 1 state at timestep -3."; pi_input_1_delayed_5 "Preprocessed initial input 1 state at timestep -4."; ai_layer_2_delayed_1 "Initial layer 2 state at timestep 0."; ai_layer_2_delayed_2 "Initial layer 2 state at timestep -1."; ai_layer_2_delayed_3 "Initial layer 2 state at timestep -2."; ai_layer_2_delayed_4 "Initial layer 2 state at timestep -3."; ai_layer_2_delayed_5 "Initial layer 2 state at timestep -4."
      mask help: NARX Neural Network
      mask Display: e = 0.06;c1 = [120 150 230]/255;c2 = ([120 150 230]+0)/383;c3 = ([120 150 230]+128)/383;patch([0 1 1 0],[0 0 1 1],c1);patch([0 1 1 1-e 1-e 0+e],[0 0 1 1-e 0+e 0+e],c2);patch([0 0 1 1-e 0+e 0+e],[0 1 1 1-e 1-e 0+e],c3);plot([0 1 1 0 0],[0 0 1 1 0]);fprintf('NNET');port_label('input',1,' x');port_label('output',1,'y ');
  Plant Neural Network 001 copy : Subsystem  Commented=on  mask{pi_input_1_delayed_1=0, pi_input_1_delayed_2=0, pi_input_1_delayed_3=0, pi_input_1_delayed_4=0, pi_input_1_delayed_5=0, ai_layer_2_delayed_1=0, ai_layer_2_delayed_2=0, ai_layer_2_delayed_3=0, ai_layer_2_delayed_4=0, ai_layer_2_delayed_5=0}
      mask prompts: pi_input_1_delayed_1 "Preprocessed initial input 1 state at timestep 0."; pi_input_1_delayed_2 "Preprocessed initial input 1 state at timestep -1."; pi_input_1_delayed_3 "Preprocessed initial input 1 state at timestep -2."; pi_input_1_delayed_4 "Preprocessed initial input 1 state at timestep -3."; pi_input_1_delayed_5 "Preprocessed initial input 1 state at timestep -4."; ai_layer_2_delayed_1 "Initial layer 2 state at timestep 0."; ai_layer_2_delayed_2 "Initial layer 2 state at timestep -1."; ai_layer_2_delayed_3 "Initial layer 2 state at timestep -2."; ai_layer_2_delayed_4 "Initial layer 2 state at timestep -3."; ai_layer_2_delayed_5 "Initial layer 2 state at timestep -4."
      mask help: NARX Neural Network
      mask Display: e = 0.06;c1 = [120 150 230]/255;c2 = ([120 150 230]+0)/383;c3 = ([120 150 230]+128)/383;patch([0 1 1 0],[0 0 1 1],c1);patch([0 1 1 1-e 1-e 0+e],[0 0 1 1-e 0+e 0+e],c2);patch([0 0 1 1-e 0+e 0+e],[0 1 1 1-e 1-e 0+e],c3);plot([0 1 1 0 0],[0 0 1 1 0]);fprintf('NNET');port_label('input',1,' x');port_label('output',1,'y ');
  Plant Neural Network 001 copy1 : Subsystem  Commented=on  mask{pi_input_1_delayed_1=0, pi_input_1_delayed_2=0, pi_input_1_delayed_3=0, pi_input_1_delayed_4=0, pi_input_1_delayed_5=0, ai_layer_2_delayed_1=0, ai_layer_2_delayed_2=0, ai_layer_2_delayed_3=0, ai_layer_2_delayed_4=0, ai_layer_2_delayed_5=0}
      mask prompts: pi_input_1_delayed_1 "Preprocessed initial input 1 state at timestep 0."; pi_input_1_delayed_2 "Preprocessed initial input 1 state at timestep -1."; pi_input_1_delayed_3 "Preprocessed initial input 1 state at timestep -2."; pi_input_1_delayed_4 "Preprocessed initial input 1 state at timestep -3."; pi_input_1_delayed_5 "Preprocessed initial input 1 state at timestep -4."; ai_layer_2_delayed_1 "Initial layer 2 state at timestep 0."; ai_layer_2_delayed_2 "Initial layer 2 state at timestep -1."; ai_layer_2_delayed_3 "Initial layer 2 state at timestep -2."; ai_layer_2_delayed_4 "Initial layer 2 state at timestep -3."; ai_layer_2_delayed_5 "Initial layer 2 state at timestep -4."
      mask help: NARX Neural Network
      mask Display: e = 0.06;c1 = [120 150 230]/255;c2 = ([120 150 230]+0)/383;c3 = ([120 150 230]+128)/383;patch([0 1 1 0],[0 0 1 1],c1);patch([0 1 1 1-e 1-e 0+e],[0 0 1 1-e 0+e 0+e],c2);patch([0 0 1 1-e 0+e 0+e],[0 1 1 1-e 1-e 0+e],c3);plot([0 1 1 0 0],[0 0 1 1 0]);fprintf('NNET');port_label('input',1,' x');port_label('output',1,'y ');
  Plant Neural Network 001 copy2 : Subsystem  Commented=on  mask{pi_input_1_delayed_1=0, pi_input_1_delayed_2=0, pi_input_1_delayed_3=0, pi_input_1_delayed_4=0, pi_input_1_delayed_5=0, ai_layer_2_delayed_1=0, ai_layer_2_delayed_2=0, ai_layer_2_delayed_3=0, ai_layer_2_delayed_4=0, ai_layer_2_delayed_5=0}
      mask prompts: pi_input_1_delayed_1 "Preprocessed initial input 1 state at timestep 0."; pi_input_1_delayed_2 "Preprocessed initial input 1 state at timestep -1."; pi_input_1_delayed_3 "Preprocessed initial input 1 state at timestep -2."; pi_input_1_delayed_4 "Preprocessed initial input 1 state at timestep -3."; pi_input_1_delayed_5 "Preprocessed initial input 1 state at timestep -4."; ai_layer_2_delayed_1 "Initial layer 2 state at timestep 0."; ai_layer_2_delayed_2 "Initial layer 2 state at timestep -1."; ai_layer_2_delayed_3 "Initial layer 2 state at timestep -2."; ai_layer_2_delayed_4 "Initial layer 2 state at timestep -3."; ai_layer_2_delayed_5 "Initial layer 2 state at timestep -4."
      mask help: NARX Neural Network
      mask Display: e = 0.06;c1 = [120 150 230]/255;c2 = ([120 150 230]+0)/383;c3 = ([120 150 230]+128)/383;patch([0 1 1 0],[0 0 1 1],c1);patch([0 1 1 1-e 1-e 0+e],[0 0 1 1-e 0+e 0+e],c2);patch([0 0 1 1-e 0+e 0+e],[0 1 1 1-e 1-e 0+e],c3);plot([0 1 1 0 0],[0 0 1 1 0]);fprintf('NNET');port_label('input',1,' x');port_label('output',1,'y ');
  Plant neural network 001 backup : Subsystem  Commented=on  mask{pi_input_1_delayed_1=0, pi_input_1_delayed_2=0, pi_input_1_delayed_3=0, pi_input_1_delayed_4=0, pi_input_1_delayed_5=0, ai_layer_2_delayed_1=0, ai_layer_2_delayed_2=0, ai_layer_2_delayed_3=0, ai_layer_2_delayed_4=0, ai_layer_2_delayed_5=0}
      mask prompts: pi_input_1_delayed_1 "Preprocessed initial input 1 state at timestep 0."; pi_input_1_delayed_2 "Preprocessed initial input 1 state at timestep -1."; pi_input_1_delayed_3 "Preprocessed initial input 1 state at timestep -2."; pi_input_1_delayed_4 "Preprocessed initial input 1 state at timestep -3."; pi_input_1_delayed_5 "Preprocessed initial input 1 state at timestep -4."; ai_layer_2_delayed_1 "Initial layer 2 state at timestep 0."; ai_layer_2_delayed_2 "Initial layer 2 state at timestep -1."; ai_layer_2_delayed_3 "Initial layer 2 state at timestep -2."; ai_layer_2_delayed_4 "Initial layer 2 state at timestep -3."; ai_layer_2_delayed_5 "Initial layer 2 state at timestep -4."
      mask help: NARX Neural Network
      mask Display: e = 0.06;c1 = [120 150 230]/255;c2 = ([120 150 230]+0)/383;c3 = ([120 150 230]+128)/383;patch([0 1 1 0],[0 0 1 1],c1);patch([0 1 1 1-e 1-e 0+e],[0 0 1 1-e 0+e 0+e],c2);patch([0 0 1 1-e 0+e 0+e],[0 1 1 1-e 1-e 0+e],c3);plot([0 1 1 0 0],[0 0 1 1 0]);fprintf('NNET');port_label('input',1,' x');port_label('output',1,'y ');
  Scope{,3,7,11,13,15,17..18,20..22} (11 alike) : Scope  Commented=on
  Scope1 : Scope  NumInputPorts=2
  Scope{2,4,6,8..10,12,14,19} (9 alike) : Scope  Commented=on  NumInputPorts=2
  Scope16 : Scope  Commented=on  NumInputPorts=3
  Scope23 : Scope
  Scope24 : Scope
  Scope5 : Scope  Commented=on  NumInputPorts=3
  Step{,2..7,10..12,14,17..18} (13 alike) : Step  Commented=on  Time=0  SampleTime=0
  Step1 : Step  Time=15  SampleTime=0
  Step13 : Step  Commented=on  Time=75  After=-0.5  SampleTime=0
  Step15 : Step  Commented=on  Time=50  After=0.6  SampleTime=0
  Step16 : Step  Commented=on  Time=50  After=0.6  SampleTime=0
  Step19 : Step  Time=0  SampleTime=0
  Step20 : Step  Time=0  SampleTime=0
  Step8 : Step  Commented=on  Time=50  After=0.6  SampleTime=0
  Step9 : Step  Commented=on  Time=0  After=5  SampleTime=0
  Sum{,1..7,10..12,14,17..18,21} (15 alike) : Sum  Commented=on  Inputs=|+-
  Sum13 : Sum  Commented=on  Inputs=|++
  Sum{8,15,19,22} (4 alike) : Sum  Commented=on  Inputs=++|
  Sum16 : Sum  Commented=on  Inputs=-+|
  Sum20 : Sum  Commented=on  Inputs=-+|
  Sum9 : Sum  Commented=on  Inputs=-+|
  Switch : Switch  Commented=on  Criteria=u2 > Threshold  Threshold=50  SaturateOnIntegerOverflow=off  InputSameDT=off
  To Workspace : ToWorkspace  Commented=on  VariableName=plant_in  SaveFormat=Timeseries  SampleTime=-1
  To Workspace1 : ToWorkspace  Commented=on  VariableName=plant_out  SaveFormat=Timeseries  SampleTime=-1
  To Workspace2 : ToWorkspace  Commented=on  VariableName=pid_in  SaveFormat=Timeseries  SampleTime=-1
  To Workspace3 : ToWorkspace  Commented=on  VariableName=pid_out  SaveFormat=Timeseries  SampleTime=-1
  To Workspace4 : ToWorkspace  Commented=on  VariableName=pid_in  SaveFormat=Timeseries  SampleTime=-1
  To Workspace5 : ToWorkspace  Commented=on  VariableName=pid_out  SaveFormat=Timeseries  SampleTime=-1
  To Workspace6 : ToWorkspace  Commented=on  VariableName=imc_c_in  SaveFormat=Timeseries  SampleTime=-1
  To Workspace7 : ToWorkspace  Commented=on  VariableName=imc_c_out  SaveFormat=Timeseries  SampleTime=-1
  To Workspace8 : ToWorkspace  Commented=on  VariableName=imc_c_in2  SaveFormat=Timeseries  SampleTime=-1
  To Workspace9 : ToWorkspace  Commented=on  VariableName=imc_c_out2  SaveFormat=Timeseries  SampleTime=-1
  Transfer Fcn{,2..8,11..12,15..23} (19 alike) : TransferFcn  Commented=on  Numerator=3  Denominator=[8 6 1]
  Transfer Fcn1 : TransferFcn  Numerator=3  Denominator=[8 6 1]
  Transfer Fcn10 : TransferFcn  Commented=on  Numerator=[8 6 1]  Denominator=3*filter_3
  Transfer Fcn13 : TransferFcn  Commented=on  Numerator=[8 6 1]  Denominator=3*filter_x
  Transfer Fcn14 : TransferFcn  Commented=on  Numerator=[8 6 1]  Denominator=3*filter_x
  Transfer Fcn24 : TransferFcn  Numerator=3  Denominator=[8 6 1]
  Transfer Fcn25 : TransferFcn  Numerator=3  Denominator=[8 6 1]
  Transfer Fcn9 : TransferFcn  Commented=on  Numerator=[8 6 1]  Denominator=3*filter_3
  Uniform Random Number{,2..5} (5 alike) : UniformRandomNumber  Commented=on  SampleTime=0.01
  Uniform Random Number1 : UniformRandomNumber  Minimum=0  SampleTime=0.05
  solution3imc2 : Subsystem  Commented=on  mask{pi_input_1_delayed_1=0, pi_input_1_delayed_2=0, pi_input_1_delayed_3=0, pi_input_1_delayed_4=0, pi_input_1_delayed_5=0, pi_input_1_delayed_6=0, ai_layer_2_delayed_1=0, ai_layer_2_delayed_2=0, ai_layer_2_delayed_3=0, ai_layer_2_delayed_4=0, ai_layer_2_delayed_5=0, ai_layer_2_delayed_6=0}
      mask prompts: pi_input_1_delayed_1 "Preprocessed initial input 1 state at timestep 0."; pi_input_1_delayed_2 "Preprocessed initial input 1 state at timestep -1."; pi_input_1_delayed_3 "Preprocessed initial input 1 state at timestep -2."; pi_input_1_delayed_4 "Preprocessed initial input 1 state at timestep -3."; pi_input_1_delayed_5 "Preprocessed initial input 1 state at timestep -4."; pi_input_1_delayed_6 "Preprocessed initial input 1 state at timestep -5."; ai_layer_2_delayed_1 "Initial layer 2 state at timestep 0."; ai_layer_2_delayed_2 "Initial layer 2 state at timestep -1."; ai_layer_2_delayed_3 "Initial layer 2 state at timestep -2."; ai_layer_2_delayed_4 "Initial layer 2 state at timestep -3."; ai_layer_2_delayed_5 "Initial layer 2 state at timestep -4."; ai_layer_2_delayed_6 "Initial layer 2 state at timestep -5."
      mask help: NARX Neural Network
      mask Display: e = 0.06;c1 = [120 150 230]/255;c2 = ([120 150 230]+0)/383;c3 = ([120 150 230]+128)/383;patch([0 1 1 0],[0 0 1 1],c1);patch([0 1 1 1-e 1-e 0+e],[0 0 1 1-e 0+e 0+e],c2);patch([0 0 1 1-e 0+e 0+e],[0 1 1 1-e 1-e 0+e],c3);plot([0 1 1 0 0],[0 0 1 1 0]);fprintf('NNET');port_label('input',1,' x');port_label('output',1,'y ');
  wires:
  Transfer Fcn/1 -> To Workspace1/1, Scope/1
  Transfer Fcn1/1 -> Scope1/1  "tf"
  Step1/1 -> Transfer Fcn1/1, Plant Neural Network 001/1(x)
  Plant Neural Network 001/1(y) -> Scope1/2  "nn"
  PID Controller1/1 -> Scope2/2, To Workspace3/1
  Step4/1 -> Sum1/1, Sum/1, Sum2/1
  Uniform Random Number2/1 -> PI Neural Network1/1(x), Filter/1, To Workspace2/1
  Sum/1 -> PID Controller/1
  PID Controller/1 -> Transfer Fcn2/1
  Transfer Fcn2/1 -> Scope5/1, Scope4/1, Sum/2, Scope3/1  "pi"
  Uniform Random Number/1 -> To Workspace/1, Transfer Fcn/1
  Filter/1 -> PID Controller1/1
  Transfer Fcn3/1 -> Scope5/2, Sum1/2, Scope4/2  "pi_f"
  PID Controller2/1 -> Transfer Fcn3/1
  Sum1/1 -> Filter1/1
  Filter1/1 -> PID Controller2/1
  Transfer Fcn4/1 -> Sum2/2, Scope5/3  "nn"
  PI Neural Network1/1(y) -> Scope2/1
  PID Neural Network/1(y) -> Transfer Fcn7/1
  Transfer Fcn7/1 -> Sum5/2, Scope8/2  "nnet"
  Filter3/1 -> PID Controller5/1
  Sum4/1 -> Filter5/1
  PID Controller5/1 -> Transfer Fcn6/1
  Transfer Fcn6/1 -> Scope8/1, Sum4/2  "pid_f"
  Filter2/1 -> PID Controller4/1
  Transfer Fcn5/1 -> Scope7/1, Sum3/2
  PID Controller3/1 -> Transfer Fcn5/1
  Sum3/1 -> PID Controller3/1
  Uniform Random Number3/1 -> Filter4/1, To Workspace4/1
  Step5/1 -> Sum4/1, Sum5/1
  PID Controller4/1 -> To Workspace5/1, Scope6/2
  Filter4/1 -> Filter2/1
  Filter5/1 -> Filter3/1
  Sum5/1 -> PID Neural Network/1(x)
  PI Neural Network/1(y) -> Transfer Fcn4/1
  Sum2/1 -> PI Neural Network/1(x)
  Transfer Fcn9/1 -> To Workspace7/1, Scope10/2
  Step6/1 -> NARX Neural Network Best1/1(x), To Workspace6/1, Transfer Fcn9/1
  Transfer Fcn10/1 -> Transfer Fcn8/1
  Transfer Fcn8/1 -> Scope12/1, Sum6/2, Scope11/1  "imc"
  Sum6/1 -> Transfer Fcn10/1
  Step7/1 -> Sum7/1, Sum6/1
  Sum7/1 -> NARX Neural Network Best/1(x)
  Transfer Fcn12/1 -> Sum7/2, Scope12/2  "nn"
  NARX Neural Network Best/1(y) -> Transfer Fcn12/1
  NARX Neural Network Best1/1(y) -> Scope10/1  "nn"
  NARX Neural Network IMC Controller/1(y) -> Plant Neural Network 001 copy/1(x), Transfer Fcn11/1
  Transfer Fcn11/1 -> Sum8/2
  Sum8/1 -> Scope13/1, Sum9/2
  Plant Neural Network 001 copy/1(y) -> Sum9/1  "nn"
  Sum10/1 -> NARX Neural Network IMC Controller/1(x)
  Sum9/1 -> Sum10/2
  Step9/1 -> Sum10/1
  NARX Neural Network IMC m9 copy1/1(y) -> Scope14/1  "nn"
  Switch/1 -> NARX Neural Network IMC m9 copy1/1(x), To Workspace8/1, Transfer Fcn13/1, Scope17/1
  Transfer Fcn13/1 -> Scope14/2, To Workspace9/1
  solution3imc2/1(y) -> Transfer Fcn15/1
  Transfer Fcn15/1 -> Scope16/2, Sum12/2  "nn3"
  Sum12/1 -> solution3imc2/1(x)
  Step10/1 -> Sum17/1, Sum12/1, Sum11/1
  Sum11/1 -> Transfer Fcn14/1
  Transfer Fcn16/1 -> Scope15/1, Sum11/2, Scope16/1
  Transfer Fcn14/1 -> Transfer Fcn16/1
  Clock/1 -> Switch/2
  Uniform Random Number5/1 -> Switch/3
  Step12/1 -> Sum13/2
  Step13/1 -> Sum13/1
  Sum13/1 -> Switch/1
  Step14/1 -> Sum14/1
  Sum16/1 -> Sum14/2
  Sum14/1 -> Hr2 Neural Network/1(x)
  Plant Neural Network 001 copy1/1(y) -> Sum16/1  "nn"
  Sum15/1 -> Sum16/2, Scope18/1
  Transfer Fcn17/1 -> Sum15/2
  Hr2 Neural Network/1(y) -> Plant Neural Network 001 copy1/1(x), Transfer Fcn17/1
  Transfer Fcn18/1 -> Scope19/1  "plant"
  NARX Neural Network m8 gud (solution 2)/1(y) -> Transfer Fcn19/1
  Transfer Fcn19/1 -> Scope16/3, Sum17/2  "nn2"
  Sum17/1 -> NARX Neural Network m8 gud (solution 2)/1(x)
  Step8/1 -> Sum15/1
  Hr2 Neural Network1/1(y) -> Transfer Fcn20/1, Plant Neural Network 001 copy2/1(x)
  Transfer Fcn20/1 -> Sum19/2
  Sum19/1 -> Scope9/1, Sum20/2  "IMC"
  Plant Neural Network 001 copy2/1(y) -> Sum20/1  "nn"
  Sum18/1 -> Hr2 Neural Network1/1(x)
  Sum20/1 -> Sum18/2
  Step11/1 -> Sum21/1, Sum18/1
  PID Neural Network1/1(y) -> Transfer Fcn21/1
  Sum21/1 -> PID Neural Network1/1(x)
  Sum22/1 -> Sum21/2, Scope9/2, Scope20/1  "PID"
  Transfer Fcn21/1 -> Sum22/2
  Step15/1 -> Sum19/1
  Step16/1 -> Sum22/1
  Model Reference Controller/1 -> Transfer Fcn22/1
  Transfer Fcn22/1 -> Model Reference Controller/2, Scope21/1
  Step17/1 -> Model Reference Controller/1
  Model Reference Controller1/1 -> Transfer Fcn23/1  "Torque"
  Transfer Fcn23/1 -> Model Reference Controller1/2, Scope22/1
  Step18/1 -> Model Reference Controller1/1
  Step19/1 -> NARMA-L2 Controller/1
  NARMA-L2 Controller/1 -> Transfer Fcn24/1  "Current"
  Transfer Fcn24/1 -> NARMA-L2 Controller/2, Scope23/1
  Transfer Fcn25/1 -> NARMA-L2 Controller1/2, Scope24/1
  NARMA-L2 Controller1/1 -> Transfer Fcn25/1
  Step20/1 -> NARMA-L2 Controller1/1
